simulink model "mux4_1_model"  (R2023b)
settings: Solver=VariableStepAuto  StartTime=0.0  StopTime=10.0  RelTol=1e-3
libraries: neural x204
(part 2 of 4)

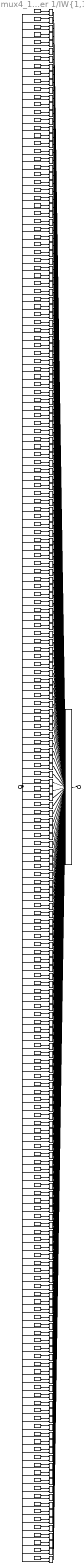
== system mux4_1_model/Pattern Recognition Neural Network/Layer 1/IW{1,1} ==
  "pd{1,1}" : Inport  PortDimensions=6
      mask Display: e = 0.06;c1 = [120 230 180]/255;c2 = ([120 230 180]+0)/(256+128);c3 = ([120 230 180]+128)/(256+128);patch([0 1 1 0],[0 0 1 1],c1);patch([0 1 1 1-e 1-e 0+e],[0 0 1 1-e 0+e 0+e],c2);patch([0 0 1 1-e 0+e 0+e],[0 1 1 1-e 1-e 0+e],c3);plot([0 1 1 0 0],[0 0 1 1 0]);
  "IW{1,1}(1,:)'" : Constant  Value=[1.88831465030217149347890881472267210483551025390625;-1.6328420936517591410819250086206011474132537841796875;-0.00712501113071774445917316853638112661428749561309814453125;0.95499304227647596743366875671199522912502288818359375;-0.8704765472023023864522883741301484405994415283203125;-1.8583799856878278067284782082424499094486236572265625]
      mask Display: e = 0.06;c1 = [120 150 230]/255;c2 = ([120 150 230]+0)/383;c3 = ([120 150 230]+128)/383;patch([0 1 1 0],[0 0 1 1],c1);patch([0 1 1 1-e 1-e 0+e],[0 0 1 1-e 0+e 0+e],c2);patch([0 0 1 1-e 0+e 0+e],[0 1 1 1-e 1-e 0+e],c3);plot([0 1 1 0 0],[0 0 1 1 0]);disp('Weights');
  "IW{1,1}(10,:)'" : Constant  Value=[-1.75938767476387436516915840911678969860076904296875;-1.1324850355018580838617481276742182672023773193359375;-2.119105979350400570382362275267951190471649169921875;0.50814743940664242050075927181751467287540435791015625;1.1338734712628728562577862248872406780719757080078125;-0.8131088091958151853333447434124536812305450439453125]
      mask Display: e = 0.06;c1 = [120 150 230]/255;c2 = ([120 150 230]+0)/383;c3 = ([120 150 230]+128)/383;patch([0 1 1 0],[0 0 1 1],c1);patch([0 1 1 1-e 1-e 0+e],[0 0 1 1-e 0+e 0+e],c2);patch([0 0 1 1-e 0+e 0+e],[0 1 1 1-e 1-e 0+e],c3);plot([0 1 1 0 0],[0 0 1 1 0]);disp('Weights');
  "IW{1,1}(100,:)'" : Constant  Value=[1.0766510821556865007408987366943620145320892333984375;2.50729854836723031752399037941358983516693115234375;-0.66792671741191711465290836713393218815326690673828125;1.2994231213573979033526484272442758083343505859375;-0.540478862160529871516700950451195240020751953125;-1.2539592132005139557549000528524629771709442138671875]
      mask Display: e = 0.06;c1 = [120 150 230]/255;c2 = ([120 150 230]+0)/383;c3 = ([120 150 230]+128)/383;patch([0 1 1 0],[0 0 1 1],c1);patch([0 1 1 1-e 1-e 0+e],[0 0 1 1-e 0+e 0+e],c2);patch([0 0 1 1-e 0+e 0+e],[0 1 1 1-e 1-e 0+e],c3);plot([0 1 1 0 0],[0 0 1 1 0]);disp('Weights');
  "IW{1,1}(101,:)'" : Constant  Value=[1.662379190191437761114912063931114971637725830078125;0.187490400635014820007739899665466509759426116943359375;-1.018279377777016492245820700190961360931396484375;-1.3995408467046546174827881259261630475521087646484375;-1.636461452276149142193162333569489419460296630859375;-1.73390509358015609819858582341112196445465087890625]
      mask Display: e = 0.06;c1 = [120 150 230]/255;c2 = ([120 150 230]+0)/383;c3 = ([120 150 230]+128)/383;patch([0 1 1 0],[0 0 1 1],c1);patch([0 1 1 1-e 1-e 0+e],[0 0 1 1-e 0+e 0+e],c2);patch([0 0 1 1-e 0+e 0+e],[0 1 1 1-e 1-e 0+e],c3);plot([0 1 1 0 0],[0 0 1 1 0]);disp('Weights');
  "IW{1,1}(102,:)'" : Constant  Value=[-1.3089337755879235647427094590966589748859405517578125;-1.9960191789693240149716757514397613704204559326171875;1.048776716022832733443692632135935127735137939453125;-1.4530345885058013610802163384505547583103179931640625;0.95098862747164381037379143890575505793094635009765625;1.3104674744980993050802453581127338111400604248046875]
      mask Display: e = 0.06;c1 = [120 150 230]/255;c2 = ([120 150 230]+0)/383;c3 = ([120 150 230]+128)/383;patch([0 1 1 0],[0 0 1 1],c1);patch([0 1 1 1-e 1-e 0+e],[0 0 1 1-e 0+e 0+e],c2);patch([0 0 1 1-e 0+e 0+e],[0 1 1 1-e 1-e 0+e],c3);plot([0 1 1 0 0],[0 0 1 1 0]);disp('Weights');
  "IW{1,1}(103,:)'" : Constant  Value=[2.034244858071051265113737827050499618053436279296875;-0.6838445544748481541574847142328508198261260986328125;0.31194926961552649213871291067334823310375213623046875;-0.9138731258806169766018001610063947737216949462890625;-2.21660641395503343886730363010428845882415771484375;-1.03046042192042275331687051220797002315521240234375]
      mask Display: e = 0.06;c1 = [120 150 230]/255;c2 = ([120 150 230]+0)/383;c3 = ([120 150 230]+128)/383;patch([0 1 1 0],[0 0 1 1],c1);patch([0 1 1 1-e 1-e 0+e],[0 0 1 1-e 0+e 0+e],c2);patch([0 0 1 1-e 0+e 0+e],[0 1 1 1-e 1-e 0+e],c3);plot([0 1 1 0 0],[0 0 1 1 0]);disp('Weights');
  "IW{1,1}(104,:)'" : Constant  Value=[1.2341260249343211086170413182117044925689697265625;1.9697753308339509548119394821696914732456207275390625;0.7954003142586156815951881071669049561023712158203125;-0.81498512744941986607472017567488364875316619873046875;-1.7842383912172545823437985745840705931186676025390625;1.27988877349261098714805484632961452007293701171875]
      mask Display: e = 0.06;c1 = [120 150 230]/255;c2 = ([120 150 230]+0)/383;c3 = ([120 150 230]+128)/383;patch([0 1 1 0],[0 0 1 1],c1);patch([0 1 1 1-e 1-e 0+e],[0 0 1 1-e 0+e 0+e],c2);patch([0 0 1 1-e 0+e 0+e],[0 1 1 1-e 1-e 0+e],c3);plot([0 1 1 0 0],[0 0 1 1 0]);disp('Weights');
  "IW{1,1}(105,:)'" : Constant  Value=[-0.6772763005036441796846702345646917819976806640625;-2.235366208999728154793729117955081164836883544921875;-1.664847534511748161634159259847365319728851318359375;1.1604986785562731999021934825577773153781890869140625;1.363475786119232591175887137069366872310638427734375;-0.038074786361743585827444036340239108540117740631103515625]
      mask Display: e = 0.06;c1 = [120 150 230]/255;c2 = ([120 150 230]+0)/383;c3 = ([120 150 230]+128)/383;patch([0 1 1 0],[0 0 1 1],c1);patch([0 1 1 1-e 1-e 0+e],[0 0 1 1-e 0+e 0+e],c2);patch([0 0 1 1-e 0+e 0+e],[0 1 1 1-e 1-e 0+e],c3);plot([0 1 1 0 0],[0 0 1 1 0]);disp('Weights');
  "IW{1,1}(106,:)'" : Constant  Value=[-1.0064124207377325159740166782285086810588836669921875;-1.85642466798463967592169865383766591548919677734375;0.51252403270238089394439384705037809908390045166015625;1.146135937560825102110584339243359863758087158203125;1.6304971971563133603666528870235197246074676513671875;-1.6941498966407813053791642232681624591350555419921875]
      mask Display: e = 0.06;c1 = [120 150 230]/255;c2 = ([120 150 230]+0)/383;c3 = ([120 150 230]+128)/383;patch([0 1 1 0],[0 0 1 1],c1);patch([0 1 1 1-e 1-e 0+e],[0 0 1 1-e 0+e 0+e],c2);patch([0 0 1 1-e 0+e 0+e],[0 1 1 1-e 1-e 0+e],c3);plot([0 1 1 0 0],[0 0 1 1 0]);disp('Weights');
  "IW{1,1}(107,:)'" : Constant  Value=[1.5111813479866660347994411495164968073368072509765625;-1.4606807787886146865474756850744597613811492919921875;0.30650959398300570146744803423644043505191802978515625;-0.31300585299283578688545048862579278647899627685546875;-1.6224966163979737121536572885815985500812530517578125;2.187239918452816400673555108369328081607818603515625]
      mask Display: e = 0.06;c1 = [120 150 230]/255;c2 = ([120 150 230]+0)/383;c3 = ([120 150 230]+128)/383;patch([0 1 1 0],[0 0 1 1],c1);patch([0 1 1 1-e 1-e 0+e],[0 0 1 1-e 0+e 0+e],c2);patch([0 0 1 1-e 0+e 0+e],[0 1 1 1-e 1-e 0+e],c3);plot([0 1 1 0 0],[0 0 1 1 0]);disp('Weights');
  "IW{1,1}(108,:)'" : Constant  Value=[-0.81530205261627630708431979655870236456394195556640625;0.670556113984504431613231645314954221248626708984375;2.113155561286254258135386407957412302494049072265625;1.2359534276509254180353991614538244903087615966796875;-1.87295706876884882063905024551786482334136962890625;-0.95610231061648665029650828728335909545421600341796875]
      mask Display: e = 0.06;c1 = [120 150 230]/255;c2 = ([120 150 230]+0)/383;c3 = ([120 150 230]+128)/383;patch([0 1 1 0],[0 0 1 1],c1);patch([0 1 1 1-e 1-e 0+e],[0 0 1 1-e 0+e 0+e],c2);patch([0 0 1 1-e 0+e 0+e],[0 1 1 1-e 1-e 0+e],c3);plot([0 1 1 0 0],[0 0 1 1 0]);disp('Weights');
  "IW{1,1}(109,:)'" : Constant  Value=[-0.436252319590053561082498845280497334897518157958984375;-0.09095977259585563690080789456260390579700469970703125;-2.019667451306033090219216319383122026920318603515625;1.135217226515316202295480252359993755817413330078125;-1.740452861528241523814131141989491879940032958984375;-1.719824326053439822459267816157080233097076416015625]
      mask Display: e = 0.06;c1 = [120 150 230]/255;c2 = ([120 150 230]+0)/383;c3 = ([120 150 230]+128)/383;patch([0 1 1 0],[0 0 1 1],c1);patch([0 1 1 1-e 1-e 0+e],[0 0 1 1-e 0+e 0+e],c2);patch([0 0 1 1-e 0+e 0+e],[0 1 1 1-e 1-e 0+e],c3);plot([0 1 1 0 0],[0 0 1 1 0]);disp('Weights');
  "IW{1,1}(11,:)'" : Constant  Value=[-1.86575481636632733994929367327131330966949462890625;0.259288778150366272523541510963696055114269256591796875;-1.8136703027089835504881421002210117876529693603515625;-0.91444566311584907225551432929933071136474609375;1.9041793386665977205751687506563030183315277099609375;-0.319398387228080171684752031069365330040454864501953125]
      mask Display: e = 0.06;c1 = [120 150 230]/255;c2 = ([120 150 230]+0)/383;c3 = ([120 150 230]+128)/383;patch([0 1 1 0],[0 0 1 1],c1);patch([0 1 1 1-e 1-e 0+e],[0 0 1 1-e 0+e 0+e],c2);patch([0 0 1 1-e 0+e 0+e],[0 1 1 1-e 1-e 0+e],c3);plot([0 1 1 0 0],[0 0 1 1 0]);disp('Weights');
  "IW{1,1}(110,:)'" : Constant  Value=[1.537058356646926693400700969505123794078826904296875;-0.9116668944426524756607932431506924331188201904296875;-1.3787755595316422141394241407397203147411346435546875;1.550419199126075842087857381557114422321319580078125;-1.0467684012883504696134195910417474806308746337890625;1.713054093403851840804463790846057236194610595703125]
      mask Display: e = 0.06;c1 = [120 150 230]/255;c2 = ([120 150 230]+0)/383;c3 = ([120 150 230]+128)/383;patch([0 1 1 0],[0 0 1 1],c1);patch([0 1 1 1-e 1-e 0+e],[0 0 1 1-e 0+e 0+e],c2);patch([0 0 1 1-e 0+e 0+e],[0 1 1 1-e 1-e 0+e],c3);plot([0 1 1 0 0],[0 0 1 1 0]);disp('Weights');
  "IW{1,1}(111,:)'" : Constant  Value=[-0.41550052784004432027131770155392587184906005859375;0.236723054659539633437503880486474372446537017822265625;1.7573231008430967303723946315585635602474212646484375;0.8226695216362298612722270263475365936756134033203125;-2.003254396611740428824077753233723342418670654296875;-1.9768638000240625895997936822823248803615570068359375]
      mask Display: e = 0.06;c1 = [120 150 230]/255;c2 = ([120 150 230]+0)/383;c3 = ([120 150 230]+128)/383;patch([0 1 1 0],[0 0 1 1],c1);patch([0 1 1 1-e 1-e 0+e],[0 0 1 1-e 0+e 0+e],c2);patch([0 0 1 1-e 0+e 0+e],[0 1 1 1-e 1-e 0+e],c3);plot([0 1 1 0 0],[0 0 1 1 0]);disp('Weights');
  "IW{1,1}(112,:)'" : Constant  Value=[-0.1553479606238077348479009742732159793376922607421875;0.70635925505895313936122192899347282946109771728515625;0.034497490565917721117017435972229577600955963134765625;-1.6002764274101297647945330027141608297824859619140625;-1.86061865188189567987819827976636588573455810546875;2.3375659489914095701124097104184329509735107421875]
      mask Display: e = 0.06;c1 = [120 150 230]/255;c2 = ([120 150 230]+0)/383;c3 = ([120 150 230]+128)/383;patch([0 1 1 0],[0 0 1 1],c1);patch([0 1 1 1-e 1-e 0+e],[0 0 1 1-e 0+e 0+e],c2);patch([0 0 1 1-e 0+e 0+e],[0 1 1 1-e 1-e 0+e],c3);plot([0 1 1 0 0],[0 0 1 1 0]);disp('Weights');
  "IW{1,1}(113,:)'" : Constant  Value=[-1.845377127149288920548997339210473001003265380859375;1.361228310922412365613354268134571611881256103515625;-0.758660517597993244720555594540201127529144287109375;-1.6822874639743139457692677751765586435794830322265625;1.095563177245159725003986750380136072635650634765625;-1.1994489528488203600176120744436047971248626708984375]
      mask Display: e = 0.06;c1 = [120 150 230]/255;c2 = ([120 150 230]+0)/383;c3 = ([120 150 230]+128)/383;patch([0 1 1 0],[0 0 1 1],c1);patch([0 1 1 1-e 1-e 0+e],[0 0 1 1-e 0+e 0+e],c2);patch([0 0 1 1-e 0+e 0+e],[0 1 1 1-e 1-e 0+e],c3);plot([0 1 1 0 0],[0 0 1 1 0]);disp('Weights');
  "IW{1,1}(114,:)'" : Constant  Value=[-1.1532348209103002734110532401246018707752227783203125;2.02574040678284550409671282977797091007232666015625;0.03595926287364765994158943840375286526978015899658203125;1.637336374892405910230763765866868197917938232421875;-1.4152723289234547809911646254477091133594512939453125;-1.342590343662893648257750101038254797458648681640625]
      mask Display: e = 0.06;c1 = [120 150 230]/255;c2 = ([120 150 230]+0)/383;c3 = ([120 150 230]+128)/383;patch([0 1 1 0],[0 0 1 1],c1);patch([0 1 1 1-e 1-e 0+e],[0 0 1 1-e 0+e 0+e],c2);patch([0 0 1 1-e 0+e 0+e],[0 1 1 1-e 1-e 0+e],c3);plot([0 1 1 0 0],[0 0 1 1 0]);disp('Weights');
  "IW{1,1}(115,:)'" : Constant  Value=[-1.5524401238853666740169501281343400478363037109375;1.666216443357559029436743003316223621368408203125;-1.082598303285360774594892063760198652744293212890625;-0.81942242561225320240936298432643525302410125732421875;-0.7656941750687067393954521321575157344341278076171875;1.9201958846802698044342605498968623578548431396484375]
      mask Display: e = 0.06;c1 = [120 150 230]/255;c2 = ([120 150 230]+0)/383;c3 = ([120 150 230]+128)/383;patch([0 1 1 0],[0 0 1 1],c1);patch([0 1 1 1-e 1-e 0+e],[0 0 1 1-e 0+e 0+e],c2);patch([0 0 1 1-e 0+e 0+e],[0 1 1 1-e 1-e 0+e],c3);plot([0 1 1 0 0],[0 0 1 1 0]);disp('Weights');
  "IW{1,1}(116,:)'" : Constant  Value=[-1.7401694103994957973924329053261317312717437744140625;1.47612141184980760755252049420960247516632080078125;-0.8518124355427427740750090379151515662670135498046875;1.5173408084150123986688640798092819750308990478515625;-0.72172092986768487943294303477159701287746429443359375;1.5888961206524860880762162196333520114421844482421875]
      mask Display: e = 0.06;c1 = [120 150 230]/255;c2 = ([120 150 230]+0)/383;c3 = ([120 150 230]+128)/383;patch([0 1 1 0],[0 0 1 1],c1);patch([0 1 1 1-e 1-e 0+e],[0 0 1 1-e 0+e 0+e],c2);patch([0 0 1 1-e 0+e 0+e],[0 1 1 1-e 1-e 0+e],c3);plot([0 1 1 0 0],[0 0 1 1 0]);disp('Weights');
  "IW{1,1}(117,:)'" : Constant  Value=[-1.899523414272333621255484104040078818798065185546875;0.155841010708632043968435709757613949477672576904296875;-2.08942613232541329892910653143189847469329833984375;1.6325415730440149264524052341585047543048858642578125;0.269439984105174501483048743466497398912906646728515625;0.8416068349956320471250137416063807904720306396484375]
      mask Display: e = 0.06;c1 = [120 150 230]/255;c2 = ([120 150 230]+0)/383;c3 = ([120 150 230]+128)/383;patch([0 1 1 0],[0 0 1 1],c1);patch([0 1 1 1-e 1-e 0+e],[0 0 1 1-e 0+e 0+e],c2);patch([0 0 1 1-e 0+e 0+e],[0 1 1 1-e 1-e 0+e],c3);plot([0 1 1 0 0],[0 0 1 1 0]);disp('Weights');
  "IW{1,1}(118,:)'" : Constant  Value=[-0.87634837696015266406135424404055811464786529541015625;-1.7801798972276754451371516552171669900417327880859375;2.0552891938640858171538638998754322528839111328125;-1.6794680704590005948517728029401041567325592041015625;-0.015750101229376957390204694320345879532396793365478515625;0.8263635683078442983884315253817476332187652587890625]
      mask Display: e = 0.06;c1 = [120 150 230]/255;c2 = ([120 150 230]+0)/383;c3 = ([120 150 230]+128)/383;patch([0 1 1 0],[0 0 1 1],c1);patch([0 1 1 1-e 1-e 0+e],[0 0 1 1-e 0+e 0+e],c2);patch([0 0 1 1-e 0+e 0+e],[0 1 1 1-e 1-e 0+e],c3);plot([0 1 1 0 0],[0 0 1 1 0]);disp('Weights');
  "IW{1,1}(119,:)'" : Constant  Value=[-1.516871482482184063655950012616813182830810546875;0.2370260290232108213448469768991344608366489410400390625;0.3801253712942063156532412904198281466960906982421875;2.412357471952862653097326983697712421417236328125;1.507165727561675883094949313090182840824127197265625;-0.929618773510952678407193161547183990478515625]
      mask Display: e = 0.06;c1 = [120 150 230]/255;c2 = ([120 150 230]+0)/383;c3 = ([120 150 230]+128)/383;patch([0 1 1 0],[0 0 1 1],c1);patch([0 1 1 1-e 1-e 0+e],[0 0 1 1-e 0+e 0+e],c2);patch([0 0 1 1-e 0+e 0+e],[0 1 1 1-e 1-e 0+e],c3);plot([0 1 1 0 0],[0 0 1 1 0]);disp('Weights');
  "IW{1,1}(12,:)'" : Constant  Value=[-0.09285344453561028554844369864440523087978363037109375;-0.1842082224482888275218783746822737157344818115234375;-2.073360096033266319892618412268348038196563720703125;-2.4221605191648567512174849980510771274566650390625;1.0905367265629186679376516622141934931278228759765625;-0.1863687345116258331501057909918017685413360595703125]
      mask Display: e = 0.06;c1 = [120 150 230]/255;c2 = ([120 150 230]+0)/383;c3 = ([120 150 230]+128)/383;patch([0 1 1 0],[0 0 1 1],c1);patch([0 1 1 1-e 1-e 0+e],[0 0 1 1-e 0+e 0+e],c2);patch([0 0 1 1-e 0+e 0+e],[0 1 1 1-e 1-e 0+e],c3);plot([0 1 1 0 0],[0 0 1 1 0]);disp('Weights');
  "IW{1,1}(120,:)'" : Constant  Value=[0.7298760298497335430312205062364228069782257080078125;1.7054105885259678299092911402112804353237152099609375;-1.3051263069442622377636098462971858680248260498046875;-1.35858548608056661777254703338257968425750732421875;1.917274474423834806913191641797311604022979736328125;0.86507265992183801639470175359747372567653656005859375]
      mask Display: e = 0.06;c1 = [120 150 230]/255;c2 = ([120 150 230]+0)/383;c3 = ([120 150 230]+128)/383;patch([0 1 1 0],[0 0 1 1],c1);patch([0 1 1 1-e 1-e 0+e],[0 0 1 1-e 0+e 0+e],c2);patch([0 0 1 1-e 0+e 0+e],[0 1 1 1-e 1-e 0+e],c3);plot([0 1 1 0 0],[0 0 1 1 0]);disp('Weights');
  "IW{1,1}(121,:)'" : Constant  Value=[-0.73181033977736176243666932350606657564640045166015625;0.312391685715092071173870635902858339250087738037109375;-0.0668938432206781230515701963668107055127620697021484375;2.07913361094917892302191830822266638278961181640625;-2.520514999819232659916679040179587900638580322265625;-0.146896648267278440158634111867286264896392822265625]
      mask Display: e = 0.06;c1 = [120 150 230]/255;c2 = ([120 150 230]+0)/383;c3 = ([120 150 230]+128)/383;patch([0 1 1 0],[0 0 1 1],c1);patch([0 1 1 1-e 1-e 0+e],[0 0 1 1-e 0+e 0+e],c2);patch([0 0 1 1-e 0+e 0+e],[0 1 1 1-e 1-e 0+e],c3);plot([0 1 1 0 0],[0 0 1 1 0]);disp('Weights');
  "IW{1,1}(122,:)'" : Constant  Value=[1.3070750508070141382432893806253559887409210205078125;-0.9616164029817337866035131810349412262439727783203125;-0.08443827552280382120475366036771447397768497467041015625;2.193825628303860408863101838505826890468597412109375;1.52403626309709494535127305425703525543212890625;-1.309713213829291955647704526199959218502044677734375]
      mask Display: e = 0.06;c1 = [120 150 230]/255;c2 = ([120 150 230]+0)/383;c3 = ([120 150 230]+128)/383;patch([0 1 1 0],[0 0 1 1],c1);patch([0 1 1 1-e 1-e 0+e],[0 0 1 1-e 0+e 0+e],c2);patch([0 0 1 1-e 0+e 0+e],[0 1 1 1-e 1-e 0+e],c3);plot([0 1 1 0 0],[0 0 1 1 0]);disp('Weights');
  "IW{1,1}(123,:)'" : Constant  Value=[-1.49923712543691944887314093648456037044525146484375;0.4244620066469833030708969090483151376247406005859375;-0.40272808530360026946226525979000143706798553466796875;-1.5141286090609884507074411885696463286876678466796875;-2.359891218442819127432130699162371456623077392578125;-1.0018908630430416462075982053647749125957489013671875]
      mask Display: e = 0.06;c1 = [120 150 230]/255;c2 = ([120 150 230]+0)/383;c3 = ([120 150 230]+128)/383;patch([0 1 1 0],[0 0 1 1],c1);patch([0 1 1 1-e 1-e 0+e],[0 0 1 1-e 0+e 0+e],c2);patch([0 0 1 1-e 0+e 0+e],[0 1 1 1-e 1-e 0+e],c3);plot([0 1 1 0 0],[0 0 1 1 0]);disp('Weights');
  "IW{1,1}(124,:)'" : Constant  Value=[1.5322902368928794647473523582448251545429229736328125;-0.11793400773590911878585529848351143300533294677734375;-0.6851081461647317016883107498870231211185455322265625;-0.2943333478712519823972115773358382284641265869140625;2.505058700623063128176681857439689338207244873046875;-1.5812466947481340628911539170076139271259307861328125]
      mask Display: e = 0.06;c1 = [120 150 230]/255;c2 = ([120 150 230]+0)/383;c3 = ([120 150 230]+128)/383;patch([0 1 1 0],[0 0 1 1],c1);patch([0 1 1 1-e 1-e 0+e],[0 0 1 1-e 0+e 0+e],c2);patch([0 0 1 1-e 0+e 0+e],[0 1 1 1-e 1-e 0+e],c3);plot([0 1 1 0 0],[0 0 1 1 0]);disp('Weights');
  "IW{1,1}(125,:)'" : Constant  Value=[-2.68677738690151812761541805230081081390380859375;-1.5401660115698267983219693633145652711391448974609375;-0.32853506182747749253536539981723763048648834228515625;0.9283880104413213540937022116850130259990692138671875;0.04234698018822520559911737336733494885265827178955078125;0.9995731367004336842541079022339545190334320068359375]
      mask Display: e = 0.06;c1 = [120 150 230]/255;c2 = ([120 150 230]+0)/383;c3 = ([120 150 230]+128)/383;patch([0 1 1 0],[0 0 1 1],c1);patch([0 1 1 1-e 1-e 0+e],[0 0 1 1-e 0+e 0+e],c2);patch([0 0 1 1-e 0+e 0+e],[0 1 1 1-e 1-e 0+e],c3);plot([0 1 1 0 0],[0 0 1 1 0]);disp('Weights');
  "IW{1,1}(126,:)'" : Constant  Value=[0.457656071818612841806128699317923747003078460693359375;2.265153444827204598510661526233889162540435791015625;0.95669467375376660012165075386292301118373870849609375;-0.096484289563831648894876025224220938980579376220703125;-1.3548035008472638640597551784594543278217315673828125;-1.9258228536002415243189034299575723707675933837890625]
      mask Display: e = 0.06;c1 = [120 150 230]/255;c2 = ([120 150 230]+0)/383;c3 = ([120 150 230]+128)/383;patch([0 1 1 0],[0 0 1 1],c1);patch([0 1 1 1-e 1-e 0+e],[0 0 1 1-e 0+e 0+e],c2);patch([0 0 1 1-e 0+e 0+e],[0 1 1 1-e 1-e 0+e],c3);plot([0 1 1 0 0],[0 0 1 1 0]);disp('Weights');
  "IW{1,1}(127,:)'" : Constant  Value=[-0.75665291597339001672395397690706886351108551025390625;1.9028383927140042342074366388260386884212493896484375;-0.2233557391700828620439978067224728874862194061279296875;-1.5112287486513700240919888528878800570964813232421875;-1.690661519385519451219579423195682466030120849609375;1.420623507139258112630386676755733788013458251953125]
      mask Display: e = 0.06;c1 = [120 150 230]/255;c2 = ([120 150 230]+0)/383;c3 = ([120 150 230]+128)/383;patch([0 1 1 0],[0 0 1 1],c1);patch([0 1 1 1-e 1-e 0+e],[0 0 1 1-e 0+e 0+e],c2);patch([0 0 1 1-e 0+e 0+e],[0 1 1 1-e 1-e 0+e],c3);plot([0 1 1 0 0],[0 0 1 1 0]);disp('Weights');
  "IW{1,1}(128,:)'" : Constant  Value=[-1.44129992615077551221247631474398076534271240234375;1.4293269426266572708072999375872313976287841796875;-2.19625833799338199270323457312770187854766845703125;0.83262127728390888936615965576493181288242340087890625;-1.0087616431711523556913334687124006450176239013671875;-0.77970252370232373539948866891791112720966339111328125]
      mask Display: e = 0.06;c1 = [120 150 230]/255;c2 = ([120 150 230]+0)/383;c3 = ([120 150 230]+128)/383;patch([0 1 1 0],[0 0 1 1],c1);patch([0 1 1 1-e 1-e 0+e],[0 0 1 1-e 0+e 0+e],c2);patch([0 0 1 1-e 0+e 0+e],[0 1 1 1-e 1-e 0+e],c3);plot([0 1 1 0 0],[0 0 1 1 0]);disp('Weights');
  "IW{1,1}(129,:)'" : Constant  Value=[-2.0977566009598209717523786821402609348297119140625;1.0927019132808697410297327223815955221652984619140625;-1.0054952010366411396802277522510848939418792724609375;-0.79642250791848656632510028430260717868804931640625;-1.93440528265185918144197785295546054840087890625;0.904870480070645299974785302765667438507080078125]
      mask Display: e = 0.06;c1 = [120 150 230]/255;c2 = ([120 150 230]+0)/383;c3 = ([120 150 230]+128)/383;patch([0 1 1 0],[0 0 1 1],c1);patch([0 1 1 1-e 1-e 0+e],[0 0 1 1-e 0+e 0+e],c2);patch([0 0 1 1-e 0+e 0+e],[0 1 1 1-e 1-e 0+e],c3);plot([0 1 1 0 0],[0 0 1 1 0]);disp('Weights');
  "IW{1,1}(13,:)'" : Constant  Value=[2.091769591013599605133777004084549844264984130859375;0.41385057928697255302807889165706001222133636474609375;1.989760868931273574133911097305826842784881591796875;1.4398635501659773350269233560538850724697113037109375;0.8120504378848452109451727665145881474018096923828125;0.292866351433269500592615486311842687427997589111328125]
      mask Display: e = 0.06;c1 = [120 150 230]/255;c2 = ([120 150 230]+0)/383;c3 = ([120 150 230]+128)/383;patch([0 1 1 0],[0 0 1 1],c1);patch([0 1 1 1-e 1-e 0+e],[0 0 1 1-e 0+e 0+e],c2);patch([0 0 1 1-e 0+e 0+e],[0 1 1 1-e 1-e 0+e],c3);plot([0 1 1 0 0],[0 0 1 1 0]);disp('Weights');
  "IW{1,1}(130,:)'" : Constant  Value=[1.642323168220304996367531202849932014942169189453125;1.6715915844030515557960825390182435512542724609375;0.07189659407978006566697359858153504319489002227783203125;0.71205568209645597743673306467826478183269500732421875;1.480426424780183491947127549792639911174774169921875;1.7738718406404625493877347253146581351757049560546875]
      mask Display: e = 0.06;c1 = [120 150 230]/255;c2 = ([120 150 230]+0)/383;c3 = ([120 150 230]+128)/383;patch([0 1 1 0],[0 0 1 1],c1);patch([0 1 1 1-e 1-e 0+e],[0 0 1 1-e 0+e 0+e],c2);patch([0 0 1 1-e 0+e 0+e],[0 1 1 1-e 1-e 0+e],c3);plot([0 1 1 0 0],[0 0 1 1 0]);disp('Weights');
  "IW{1,1}(131,:)'" : Constant  Value=[1.1561621493425373596863892089459113776683807373046875;0.70996729571562033900278265718952752649784088134765625;0.65702249406333346204434064929955638945102691650390625;1.7389816541611187172833297154284082353115081787109375;-1.6145127293904806276003682796726934611797332763671875;1.8873230443673689737948961919755674898624420166015625]
      mask Display: e = 0.06;c1 = [120 150 230]/255;c2 = ([120 150 230]+0)/383;c3 = ([120 150 230]+128)/383;patch([0 1 1 0],[0 0 1 1],c1);patch([0 1 1 1-e 1-e 0+e],[0 0 1 1-e 0+e 0+e],c2);patch([0 0 1 1-e 0+e 0+e],[0 1 1 1-e 1-e 0+e],c3);plot([0 1 1 0 0],[0 0 1 1 0]);disp('Weights');
  "IW{1,1}(132,:)'" : Constant  Value=[1.3500591886800383800704139503068290650844573974609375;-1.66564321719388797049532513483427464962005615234375;-0.86416547251374209448471219729981385171413421630859375;0.418297532000039662403167994852992706000804901123046875;-0.636674882782167106398674150113947689533233642578125;2.29176104609416864121840262669138610363006591796875]
      mask Display: e = 0.06;c1 = [120 150 230]/255;c2 = ([120 150 230]+0)/383;c3 = ([120 150 230]+128)/383;patch([0 1 1 0],[0 0 1 1],c1);patch([0 1 1 1-e 1-e 0+e],[0 0 1 1-e 0+e 0+e],c2);patch([0 0 1 1-e 0+e 0+e],[0 1 1 1-e 1-e 0+e],c3);plot([0 1 1 0 0],[0 0 1 1 0]);disp('Weights');
  "IW{1,1}(133,:)'" : Constant  Value=[1.7562502929443386534558158018626272678375244140625;1.4179403797342262638636611882247962057590484619140625;-0.58888339131365607936885453455033712089061737060546875;-1.5084478552824738262216897055623121559619903564453125;-1.368012614763485235158668729127384722232818603515625;1.329596182580093710612345603294670581817626953125]
      mask Display: e = 0.06;c1 = [120 150 230]/255;c2 = ([120 150 230]+0)/383;c3 = ([120 150 230]+128)/383;patch([0 1 1 0],[0 0 1 1],c1);patch([0 1 1 1-e 1-e 0+e],[0 0 1 1-e 0+e 0+e],c2);patch([0 0 1 1-e 0+e 0+e],[0 1 1 1-e 1-e 0+e],c3);plot([0 1 1 0 0],[0 0 1 1 0]);disp('Weights');
  "IW{1,1}(134,:)'" : Constant  Value=[-1.058495654154327336726737485150806605815887451171875;-1.4114962887591586682134447983116842806339263916015625;-2.220444979734403911919571328326128423213958740234375;0.372784392207425152587774164203437976539134979248046875;1.7349297171019502084021723931073211133480072021484375;-0.6071887885852900179628477417281828820705413818359375]
      mask Display: e = 0.06;c1 = [120 150 230]/255;c2 = ([120 150 230]+0)/383;c3 = ([120 150 230]+128)/383;patch([0 1 1 0],[0 0 1 1],c1);patch([0 1 1 1-e 1-e 0+e],[0 0 1 1-e 0+e 0+e],c2);patch([0 0 1 1-e 0+e 0+e],[0 1 1 1-e 1-e 0+e],c3);plot([0 1 1 0 0],[0 0 1 1 0]);disp('Weights');
  "IW{1,1}(135,:)'" : Constant  Value=[-0.92881518491902903544854552819742821156978607177734375;2.063776476347365385066723320051096379756927490234375;1.115820184186749219890089079854078590869903564453125;1.88853050385999399196634840336628258228302001953125;-0.64429482327307907585378643489093519747257232666015625;-1.10686921874346300143088228651322424411773681640625]
      mask Display: e = 0.06;c1 = [120 150 230]/255;c2 = ([120 150 230]+0)/383;c3 = ([120 150 230]+128)/383;patch([0 1 1 0],[0 0 1 1],c1);patch([0 1 1 1-e 1-e 0+e],[0 0 1 1-e 0+e 0+e],c2);patch([0 0 1 1-e 0+e 0+e],[0 1 1 1-e 1-e 0+e],c3);plot([0 1 1 0 0],[0 0 1 1 0]);disp('Weights');
  "IW{1,1}(136,:)'" : Constant  Value=[2.036609164391787629710961482487618923187255859375;-0.1280157127676240513824978961565648205578327178955078125;-0.263202182254216487944376012819702737033367156982421875;-0.79729874233306385900021950874361209571361541748046875;2.543881563311895632750747608952224254608154296875;-0.30282514188475440075620781499310396611690521240234375]
      mask Display: e = 0.06;c1 = [120 150 230]/255;c2 = ([120 150 230]+0)/383;c3 = ([120 150 230]+128)/383;patch([0 1 1 0],[0 0 1 1],c1);patch([0 1 1 1-e 1-e 0+e],[0 0 1 1-e 0+e 0+e],c2);patch([0 0 1 1-e 0+e 0+e],[0 1 1 1-e 1-e 0+e],c3);plot([0 1 1 0 0],[0 0 1 1 0]);disp('Weights');
  "IW{1,1}(137,:)'" : Constant  Value=[-0.5037815361707365102716948968009091913700103759765625;0.815746113997100952275332019780762493610382080078125;0.38447320404987639363980633788742125034332275390625;2.3893817298616593092219773097895085811614990234375;-2.083522374996051862439117030589841306209564208984375;-0.4991731637154857015303832667996175587177276611328125]
      mask Display: e = 0.06;c1 = [120 150 230]/255;c2 = ([120 150 230]+0)/383;c3 = ([120 150 230]+128)/383;patch([0 1 1 0],[0 0 1 1],c1);patch([0 1 1 1-e 1-e 0+e],[0 0 1 1-e 0+e 0+e],c2);patch([0 0 1 1-e 0+e 0+e],[0 1 1 1-e 1-e 0+e],c3);plot([0 1 1 0 0],[0 0 1 1 0]);disp('Weights');
  "IW{1,1}(138,:)'" : Constant  Value=[-0.1461107710609940435464437769041978754103183746337890625;1.1830069221112140542828683464904315769672393798828125;0.34958795177155665978574461405514739453792572021484375;-3.12225419745804888549400857300497591495513916015625;0.3209669389391738292260924936272203922271728515625;-0.28800515491499112386009073816239833831787109375]
      mask Display: e = 0.06;c1 = [120 150 230]/255;c2 = ([120 150 230]+0)/383;c3 = ([120 150 230]+128)/383;patch([0 1 1 0],[0 0 1 1],c1);patch([0 1 1 1-e 1-e 0+e],[0 0 1 1-e 0+e 0+e],c2);patch([0 0 1 1-e 0+e 0+e],[0 1 1 1-e 1-e 0+e],c3);plot([0 1 1 0 0],[0 0 1 1 0]);disp('Weights');
  "IW{1,1}(139,:)'" : Constant  Value=[1.1617009772980677606568633564165793359279632568359375;-2.081156082091216941165612297481857240200042724609375;0.6929679164687405634737160653457976877689361572265625;0.09026726970409222616797961791235138662159442901611328125;-1.619637926752290457699245962430723011493682861328125;-1.8956215286323845337079774253652431070804595947265625]
      mask Display: e = 0.06;c1 = [120 150 230]/255;c2 = ([120 150 230]+0)/383;c3 = ([120 150 230]+128)/383;patch([0 1 1 0],[0 0 1 1],c1);patch([0 1 1 1-e 1-e 0+e],[0 0 1 1-e 0+e 0+e],c2);patch([0 0 1 1-e 0+e 0+e],[0 1 1 1-e 1-e 0+e],c3);plot([0 1 1 0 0],[0 0 1 1 0]);disp('Weights');
  "IW{1,1}(14,:)'" : Constant  Value=[0.130370910445221699358597788886982016265392303466796875;0.06595470879224892002401503532382776029407978057861328125;0.93778329616634292786869764313451014459133148193359375;-2.06969875084817456212249453528784215450286865234375;1.4934974278543702297383788391016423702239990234375;1.88755523690793847180202646995894610881805419921875]
      mask Display: e = 0.06;c1 = [120 150 230]/255;c2 = ([120 150 230]+0)/383;c3 = ([120 150 230]+128)/383;patch([0 1 1 0],[0 0 1 1],c1);patch([0 1 1 1-e 1-e 0+e],[0 0 1 1-e 0+e 0+e],c2);patch([0 0 1 1-e 0+e 0+e],[0 1 1 1-e 1-e 0+e],c3);plot([0 1 1 0 0],[0 0 1 1 0]);disp('Weights');
  "IW{1,1}(140,:)'" : Constant  Value=[-1.5668111318511872553926878026686608791351318359375;-1.8963900555458652608109559878357686102390289306640625;-0.09058730954043255068075524150117416866123676300048828125;2.00894296069608646604365276289172470569610595703125;-1.1076115689669041586284947698004543781280517578125;-0.68337109145663121889668900621472857892513275146484375]
      mask Display: e = 0.06;c1 = [120 150 230]/255;c2 = ([120 150 230]+0)/383;c3 = ([120 150 230]+128)/383;patch([0 1 1 0],[0 0 1 1],c1);patch([0 1 1 1-e 1-e 0+e],[0 0 1 1-e 0+e 0+e],c2);patch([0 0 1 1-e 0+e 0+e],[0 1 1 1-e 1-e 0+e],c3);plot([0 1 1 0 0],[0 0 1 1 0]);disp('Weights');
  "IW{1,1}(141,:)'" : Constant  Value=[-0.493181477548115976272669058744213543832302093505859375;-1.5325804228412633900546779841533862054347991943359375;-2.771100199064796765213714024866931140422821044921875;-0.057448910909267451863069453565913136117160320281982421875;0.86324146711337246262729649970424361526966094970703125;-0.85581749069124446460676836068159900605678558349609375]
      mask Display: e = 0.06;c1 = [120 150 230]/255;c2 = ([120 150 230]+0)/383;c3 = ([120 150 230]+128)/383;patch([0 1 1 0],[0 0 1 1],c1);patch([0 1 1 1-e 1-e 0+e],[0 0 1 1-e 0+e 0+e],c2);patch([0 0 1 1-e 0+e 0+e],[0 1 1 1-e 1-e 0+e],c3);plot([0 1 1 0 0],[0 0 1 1 0]);disp('Weights');
  "IW{1,1}(142,:)'" : Constant  Value=[-1.197002594050322610286229974008165299892425537109375;-2.06012164904401284815094186342321336269378662109375;-0.55514828096147506020230366630130447447299957275390625;-0.72939387634823338313339036176330409944057464599609375;2.17964632194250729213536033057607710361480712890625;-0.331769298810621615647420412642532028257846832275390625]
      mask Display: e = 0.06;c1 = [120 150 230]/255;c2 = ([120 150 230]+0)/383;c3 = ([120 150 230]+128)/383;patch([0 1 1 0],[0 0 1 1],c1);patch([0 1 1 1-e 1-e 0+e],[0 0 1 1-e 0+e 0+e],c2);patch([0 0 1 1-e 0+e 0+e],[0 1 1 1-e 1-e 0+e],c3);plot([0 1 1 0 0],[0 0 1 1 0]);disp('Weights');
  "IW{1,1}(143,:)'" : Constant  Value=[-1.89530879134973506694450406939722597599029541015625;0.78522114584999991304670174940838478505611419677734375;-1.62981252929749498292721909820102155208587646484375;-0.0217639011993176027803809091665243613533675670623779296875;1.4427206524186149128041734002181328833103179931640625;-1.6263689841685760040235209089587442576885223388671875]
      mask Display: e = 0.06;c1 = [120 150 230]/255;c2 = ([120 150 230]+0)/383;c3 = ([120 150 230]+128)/383;patch([0 1 1 0],[0 0 1 1],c1);patch([0 1 1 1-e 1-e 0+e],[0 0 1 1-e 0+e 0+e],c2);patch([0 0 1 1-e 0+e 0+e],[0 1 1 1-e 1-e 0+e],c3);plot([0 1 1 0 0],[0 0 1 1 0]);disp('Weights');
  "IW{1,1}(144,:)'" : Constant  Value=[1.8842090238854665162904211683780886232852935791015625;-0.6075292780804424364049509676988236606121063232421875;-1.9113951015001158229011934963637031614780426025390625;0.0974919111882766864507487980517907999455928802490234375;1.9049949416639415655794209669693373143672943115234375;0.724713253659541312146075142663903534412384033203125]
      mask Display: e = 0.06;c1 = [120 150 230]/255;c2 = ([120 150 230]+0)/383;c3 = ([120 150 230]+128)/383;patch([0 1 1 0],[0 0 1 1],c1);patch([0 1 1 1-e 1-e 0+e],[0 0 1 1-e 0+e 0+e],c2);patch([0 0 1 1-e 0+e 0+e],[0 1 1 1-e 1-e 0+e],c3);plot([0 1 1 0 0],[0 0 1 1 0]);disp('Weights');
  "IW{1,1}(145,:)'" : Constant  Value=[0.41305865362062810230980858250404708087444305419921875;0.356846198652678359142242925372556783258914947509765625;-1.2114844952700967173342405658331699669361114501953125;2.045676916575862147595898932195268571376800537109375;0.741817205974896420883624159614555537700653076171875;-2.263235575806954447131147389882244169712066650390625]
      mask Display: e = 0.06;c1 = [120 150 230]/255;c2 = ([120 150 230]+0)/383;c3 = ([120 150 230]+128)/383;patch([0 1 1 0],[0 0 1 1],c1);patch([0 1 1 1-e 1-e 0+e],[0 0 1 1-e 0+e 0+e],c2);patch([0 0 1 1-e 0+e 0+e],[0 1 1 1-e 1-e 0+e],c3);plot([0 1 1 0 0],[0 0 1 1 0]);disp('Weights');
  "IW{1,1}(146,:)'" : Constant  Value=[-0.9008574792966952404782432495267130434513092041015625;-2.319392326746150700955695356242358684539794921875;-1.055815889789439854240526983630843460559844970703125;-1.0826923083773867251267120082047767937183380126953125;0.420690200351257315158903793417266570031642913818359375;1.71475202633863954559956255252473056316375732421875]
      mask Display: e = 0.06;c1 = [120 150 230]/255;c2 = ([120 150 230]+0)/383;c3 = ([120 150 230]+128)/383;patch([0 1 1 0],[0 0 1 1],c1);patch([0 1 1 1-e 1-e 0+e],[0 0 1 1-e 0+e 0+e],c2);patch([0 0 1 1-e 0+e 0+e],[0 1 1 1-e 1-e 0+e],c3);plot([0 1 1 0 0],[0 0 1 1 0]);disp('Weights');
  "IW{1,1}(147,:)'" : Constant  Value=[-1.8657348896215013578370189861743710935115814208984375;-1.808173279651605458440144502674229443073272705078125;-1.356709286650181756073152428143657743930816650390625;0.6217501894101615800281024348805658519268035888671875;1.238465600404463629047313588671386241912841796875;-0.9240999480794018783313958920189179480075836181640625]
      mask Display: e = 0.06;c1 = [120 150 230]/255;c2 = ([120 150 230]+0)/383;c3 = ([120 150 230]+128)/383;patch([0 1 1 0],[0 0 1 1],c1);patch([0 1 1 1-e 1-e 0+e],[0 0 1 1-e 0+e 0+e],c2);patch([0 0 1 1-e 0+e 0+e],[0 1 1 1-e 1-e 0+e],c3);plot([0 1 1 0 0],[0 0 1 1 0]);disp('Weights');
  "IW{1,1}(148,:)'" : Constant  Value=[1.3273967969385098708556824931292794644832611083984375;1.602140748976784490054114939994178712368011474609375;2.355541506071918700371270460891537368297576904296875;0.5700044310759844190528156104846857488155364990234375;-0.95792229277017149069450852039153687655925750732421875;-0.03538063002234291543057764783952734433114528656005859375]
      mask Display: e = 0.06;c1 = [120 150 230]/255;c2 = ([120 150 230]+0)/383;c3 = ([120 150 230]+128)/383;patch([0 1 1 0],[0 0 1 1],c1);patch([0 1 1 1-e 1-e 0+e],[0 0 1 1-e 0+e 0+e],c2);patch([0 0 1 1-e 0+e 0+e],[0 1 1 1-e 1-e 0+e],c3);plot([0 1 1 0 0],[0 0 1 1 0]);disp('Weights');
  "IW{1,1}(149,:)'" : Constant  Value=[1.823832672938071386425917808082886040210723876953125;-1.7778507285522879843853161219158209860324859619140625;0.40863846088071842377331677198526449501514434814453125;-1.025007037315884161898793536238372325897216796875;1.140130686179925856293948527309112250804901123046875;-1.55655716652775932828944860375486314296722412109375]
      mask Display: e = 0.06;c1 = [120 150 230]/255;c2 = ([120 150 230]+0)/383;c3 = ([120 150 230]+128)/383;patch([0 1 1 0],[0 0 1 1],c1);patch([0 1 1 1-e 1-e 0+e],[0 0 1 1-e 0+e 0+e],c2);patch([0 0 1 1-e 0+e 0+e],[0 1 1 1-e 1-e 0+e],c3);plot([0 1 1 0 0],[0 0 1 1 0]);disp('Weights');
  "IW{1,1}(15,:)'" : Constant  Value=[-1.324881363200605566277090474613942205905914306640625;1.1536904791992099728048515316913835704326629638671875;-1.6016606635338386244171715588890947401523590087890625;0.57955185806468445530725830394658260047435760498046875;-2.335715701038534319877726375125348567962646484375;-0.1892873599881935986477543565342784859240055084228515625]
      mask Display: e = 0.06;c1 = [120 150 230]/255;c2 = ([120 150 230]+0)/383;c3 = ([120 150 230]+128)/383;patch([0 1 1 0],[0 0 1 1],c1);patch([0 1 1 1-e 1-e 0+e],[0 0 1 1-e 0+e 0+e],c2);patch([0 0 1 1-e 0+e 0+e],[0 1 1 1-e 1-e 0+e],c3);plot([0 1 1 0 0],[0 0 1 1 0]);disp('Weights');
  "IW{1,1}(150,:)'" : Constant  Value=[-2.371878147957687144042893123696558177471160888671875;0.0655044238850235049920200935957836918532848358154296875;1.0935592820533523994441793547593988478183746337890625;-1.664281943452273981876032848958857357501983642578125;-1.1107501073379155709375254446058534085750579833984375;0.86158354777594248208316685122554190456867218017578125]
      mask Display: e = 0.06;c1 = [120 150 230]/255;c2 = ([120 150 230]+0)/383;c3 = ([120 150 230]+128)/383;patch([0 1 1 0],[0 0 1 1],c1);patch([0 1 1 1-e 1-e 0+e],[0 0 1 1-e 0+e 0+e],c2);patch([0 0 1 1-e 0+e 0+e],[0 1 1 1-e 1-e 0+e],c3);plot([0 1 1 0 0],[0 0 1 1 0]);disp('Weights');
  "IW{1,1}(151,:)'" : Constant  Value=[1.195318942968249142921877137268893420696258544921875;-1.8334460053959091840880546442349441349506378173828125;0.1462588780386397668831222063090535812079906463623046875;-2.505645663401897760280689908540807664394378662109375;0.40232850050565016619685820842278189957141876220703125;0.43693649941245238377263149232021532952785491943359375]
      mask Display: e = 0.06;c1 = [120 150 230]/255;c2 = ([120 150 230]+0)/383;c3 = ([120 150 230]+128)/383;patch([0 1 1 0],[0 0 1 1],c1);patch([0 1 1 1-e 1-e 0+e],[0 0 1 1-e 0+e 0+e],c2);patch([0 0 1 1-e 0+e 0+e],[0 1 1 1-e 1-e 0+e],c3);plot([0 1 1 0 0],[0 0 1 1 0]);disp('Weights');
  "IW{1,1}(152,:)'" : Constant  Value=[1.74354932998822231837721119518391788005828857421875;1.0705548463252385626987006617127917706966400146484375;-0.70414634964965883145993075231672264635562896728515625;0.2078102812847431313247881234929081983864307403564453125;2.150747726622813882357831971603445708751678466796875;-1.5889491793305208222619739899528212845325469970703125]
      mask Display: e = 0.06;c1 = [120 150 230]/255;c2 = ([120 150 230]+0)/383;c3 = ([120 150 230]+128)/383;patch([0 1 1 0],[0 0 1 1],c1);patch([0 1 1 1-e 1-e 0+e],[0 0 1 1-e 0+e 0+e],c2);patch([0 0 1 1-e 0+e 0+e],[0 1 1 1-e 1-e 0+e],c3);plot([0 1 1 0 0],[0 0 1 1 0]);disp('Weights');
  "IW{1,1}(153,:)'" : Constant  Value=[1.90366393196154692901700400398112833499908447265625;0.2834736693426476161761229377589188516139984130859375;0.19353842037546475918219357481575571000576019287109375;0.8288521409726381516946958072367124259471893310546875;0.63140449741232196334550508254324086010456085205078125;-2.557226012769431289228805326274596154689788818359375]
      mask Display: e = 0.06;c1 = [120 150 230]/255;c2 = ([120 150 230]+0)/383;c3 = ([120 150 230]+128)/383;patch([0 1 1 0],[0 0 1 1],c1);patch([0 1 1 1-e 1-e 0+e],[0 0 1 1-e 0+e 0+e],c2);patch([0 0 1 1-e 0+e 0+e],[0 1 1 1-e 1-e 0+e],c3);plot([0 1 1 0 0],[0 0 1 1 0]);disp('Weights');
  "IW{1,1}(154,:)'" : Constant  Value=[1.9977276479975056844295977498404681682586669921875;1.7548951916726165389803782090893946588039398193359375;-0.82191519881507424383215720808948390185832977294921875;-0.70626412948527106383522777832695282995700836181640625;-1.7409803629414941639197422773577272891998291015625;0.014657775493403475686182702020232682116329669952392578125]
      mask Display: e = 0.06;c1 = [120 150 230]/255;c2 = ([120 150 230]+0)/383;c3 = ([120 150 230]+128)/383;patch([0 1 1 0],[0 0 1 1],c1);patch([0 1 1 1-e 1-e 0+e],[0 0 1 1-e 0+e 0+e],c2);patch([0 0 1 1-e 0+e 0+e],[0 1 1 1-e 1-e 0+e],c3);plot([0 1 1 0 0],[0 0 1 1 0]);disp('Weights');
  "IW{1,1}(155,:)'" : Constant  Value=[1.8995122857974358066002196210320107638835906982421875;1.5043736154819209449584604953997768461704254150390625;0.606161129636155759925486563588492572307586669921875;-1.5373536548326269812747568721533752977848052978515625;-1.591438178414662285575786881963722407817840576171875;0.06951624823206754844040489160761353559792041778564453125]
      mask Display: e = 0.06;c1 = [120 150 230]/255;c2 = ([120 150 230]+0)/383;c3 = ([120 150 230]+128)/383;patch([0 1 1 0],[0 0 1 1],c1);patch([0 1 1 1-e 1-e 0+e],[0 0 1 1-e 0+e 0+e],c2);patch([0 0 1 1-e 0+e 0+e],[0 1 1 1-e 1-e 0+e],c3);plot([0 1 1 0 0],[0 0 1 1 0]);disp('Weights');
  "IW{1,1}(156,:)'" : Constant  Value=[-1.432272400282839530660794480354525148868560791015625;0.7148856169267936433442400812054984271526336669921875;1.91126977572871936672527226619422435760498046875;-1.4156832976934021761650228654616512358188629150390625;-1.43152917145521740849289926700294017791748046875;1.172722304933671910731618481804616749286651611328125]
      mask Display: e = 0.06;c1 = [120 150 230]/255;c2 = ([120 150 230]+0)/383;c3 = ([120 150 230]+128)/383;patch([0 1 1 0],[0 0 1 1],c1);patch([0 1 1 1-e 1-e 0+e],[0 0 1 1-e 0+e 0+e],c2);patch([0 0 1 1-e 0+e 0+e],[0 1 1 1-e 1-e 0+e],c3);plot([0 1 1 0 0],[0 0 1 1 0]);disp('Weights');
  "IW{1,1}(157,:)'" : Constant  Value=[0.82514023174911221847338538282201625406742095947265625;0.757110900603036096612186156562529504299163818359375;0.65557760546125887213264604724827222526073455810546875;-2.323048736401905234316700443741865456104278564453125;1.61220011486059622285438308608718216419219970703125;1.3432756129062823902131640352308750152587890625]
      mask Display: e = 0.06;c1 = [120 150 230]/255;c2 = ([120 150 230]+0)/383;c3 = ([120 150 230]+128)/383;patch([0 1 1 0],[0 0 1 1],c1);patch([0 1 1 1-e 1-e 0+e],[0 0 1 1-e 0+e 0+e],c2);patch([0 0 1 1-e 0+e 0+e],[0 1 1 1-e 1-e 0+e],c3);plot([0 1 1 0 0],[0 0 1 1 0]);disp('Weights');
  "IW{1,1}(158,:)'" : Constant  Value=[0.38374726574355821906436858625966124236583709716796875;2.428868757170236758469172855257056653499603271484375;0.54408138779493808723231040858081541955471038818359375;-1.23259760738301427096530460403300821781158447265625;-1.0722200840054967319048273566295392811298370361328125;-1.586090176180915189974029999575577676296234130859375]
      mask Display: e = 0.06;c1 = [120 150 230]/255;c2 = ([120 150 230]+0)/383;c3 = ([120 150 230]+128)/383;patch([0 1 1 0],[0 0 1 1],c1);patch([0 1 1 1-e 1-e 0+e],[0 0 1 1-e 0+e 0+e],c2);patch([0 0 1 1-e 0+e 0+e],[0 1 1 1-e 1-e 0+e],c3);plot([0 1 1 0 0],[0 0 1 1 0]);disp('Weights');
  "IW{1,1}(159,:)'" : Constant  Value=[-0.7914305279780506907627568580210208892822265625;0.47132121317842023966449005456524901092052459716796875;1.44208858715752352708250327850691974163055419921875;0.476617860247140645579833062583929859101772308349609375;-2.619735993718328881385559725458733737468719482421875;-1.1950057997358201067328309363801963627338409423828125]
      mask Display: e = 0.06;c1 = [120 150 230]/255;c2 = ([120 150 230]+0)/383;c3 = ([120 150 230]+128)/383;patch([0 1 1 0],[0 0 1 1],c1);patch([0 1 1 1-e 1-e 0+e],[0 0 1 1-e 0+e 0+e],c2);patch([0 0 1 1-e 0+e 0+e],[0 1 1 1-e 1-e 0+e],c3);plot([0 1 1 0 0],[0 0 1 1 0]);disp('Weights');
  "IW{1,1}(16,:)'" : Constant  Value=[-2.182584653355827075671413695090450346469879150390625;0.53292843233945574876742057313094846904277801513671875;-0.7324047339933541511669545798213221132755279541015625;1.2989992312042513145087241355213336646556854248046875;1.8509114306297467233974884948111139237880706787109375;0.84096746626827989512520389325800351798534393310546875]
      mask Display: e = 0.06;c1 = [120 150 230]/255;c2 = ([120 150 230]+0)/383;c3 = ([120 150 230]+128)/383;patch([0 1 1 0],[0 0 1 1],c1);patch([0 1 1 1-e 1-e 0+e],[0 0 1 1-e 0+e 0+e],c2);patch([0 0 1 1-e 0+e 0+e],[0 1 1 1-e 1-e 0+e],c3);plot([0 1 1 0 0],[0 0 1 1 0]);disp('Weights');
  "IW{1,1}(160,:)'" : Constant  Value=[0.1992861304654575393957571805003681220114231109619140625;-0.12307620847451239409764411902870051562786102294921875;0.52620993961508777392310776122030802071094512939453125;-0.7733096234141978442266918136738240718841552734375;2.730408771552901736612284366856329143047332763671875;-1.70247180339769510482028636033646762371063232421875]
      mask Display: e = 0.06;c1 = [120 150 230]/255;c2 = ([120 150 230]+0)/383;c3 = ([120 150 230]+128)/383;patch([0 1 1 0],[0 0 1 1],c1);patch([0 1 1 1-e 1-e 0+e],[0 0 1 1-e 0+e 0+e],c2);patch([0 0 1 1-e 0+e 0+e],[0 1 1 1-e 1-e 0+e],c3);plot([0 1 1 0 0],[0 0 1 1 0]);disp('Weights');
  "IW{1,1}(161,:)'" : Constant  Value=[1.2561145465200826976115422439761459827423095703125;0.7536662954489461441198727698065340518951416015625;1.69713449376881353458657031296752393245697021484375;-1.6434524699531518621142822667025029659271240234375;-1.6044760405030047412111571247805841267108917236328125;1.163716630696929765775848863995634019374847412109375]
      mask Display: e = 0.06;c1 = [120 150 230]/255;c2 = ([120 150 230]+0)/383;c3 = ([120 150 230]+128)/383;patch([0 1 1 0],[0 0 1 1],c1);patch([0 1 1 1-e 1-e 0+e],[0 0 1 1-e 0+e 0+e],c2);patch([0 0 1 1-e 0+e 0+e],[0 1 1 1-e 1-e 0+e],c3);plot([0 1 1 0 0],[0 0 1 1 0]);disp('Weights');
  "IW{1,1}(162,:)'" : Constant  Value=[-1.393618397515708817735458069364540278911590576171875;1.7802812511310273091424960512085817754268646240234375;0.67988738083755162477928024600259959697723388671875;-0.7051085406843842218194140514242462813854217529296875;1.7997269094511076925613224375410936772823333740234375;-1.4560033155896341394708315419848076999187469482421875]
      mask Display: e = 0.06;c1 = [120 150 230]/255;c2 = ([120 150 230]+0)/383;c3 = ([120 150 230]+128)/383;patch([0 1 1 0],[0 0 1 1],c1);patch([0 1 1 1-e 1-e 0+e],[0 0 1 1-e 0+e 0+e],c2);patch([0 0 1 1-e 0+e 0+e],[0 1 1 1-e 1-e 0+e],c3);plot([0 1 1 0 0],[0 0 1 1 0]);disp('Weights');
  "IW{1,1}(163,:)'" : Constant  Value=[2.36690799940245266697047554771415889263153076171875;-1.8830082419537854665492204730981029570102691650390625;-1.25677372203648918258522826363332569599151611328125;0.56294322916407402157545902809943072497844696044921875;0.44223548819071056836804700651555322110652923583984375;0.2315730932366526773069637101798434741795063018798828125]
      mask Display: e = 0.06;c1 = [120 150 230]/255;c2 = ([120 150 230]+0)/383;c3 = ([120 150 230]+128)/383;patch([0 1 1 0],[0 0 1 1],c1);patch([0 1 1 1-e 1-e 0+e],[0 0 1 1-e 0+e 0+e],c2);patch([0 0 1 1-e 0+e 0+e],[0 1 1 1-e 1-e 0+e],c3);plot([0 1 1 0 0],[0 0 1 1 0]);disp('Weights');
  "IW{1,1}(164,:)'" : Constant  Value=[0.62227996745830249647468690454843454062938690185546875;-1.757715537463049759736577470903284847736358642578125;-1.634668506778918395383470851811580359935760498046875;1.9413361169953484708372570821666158735752105712890625;0.0175177616589151895210019205251228413544595241546630859375;-1.2101222891833287587104450722108595073223114013671875]
      mask Display: e = 0.06;c1 = [120 150 230]/255;c2 = ([120 150 230]+0)/383;c3 = ([120 150 230]+128)/383;patch([0 1 1 0],[0 0 1 1],c1);patch([0 1 1 1-e 1-e 0+e],[0 0 1 1-e 0+e 0+e],c2);patch([0 0 1 1-e 0+e 0+e],[0 1 1 1-e 1-e 0+e],c3);plot([0 1 1 0 0],[0 0 1 1 0]);disp('Weights');
  "IW{1,1}(165,:)'" : Constant  Value=[0.1928854935379941959450178501356276683509349822998046875;1.6690556049158520313113740485277958214282989501953125;1.5230442642565533706289215842843987047672271728515625;1.9745224963000733708895495510660111904144287109375;-1.4326377401043546289116648040362633764743804931640625;0.63842207313354892850298938355990685522556304931640625]
      mask Display: e = 0.06;c1 = [120 150 230]/255;c2 = ([120 150 230]+0)/383;c3 = ([120 150 230]+128)/383;patch([0 1 1 0],[0 0 1 1],c1);patch([0 1 1 1-e 1-e 0+e],[0 0 1 1-e 0+e 0+e],c2);patch([0 0 1 1-e 0+e 0+e],[0 1 1 1-e 1-e 0+e],c3);plot([0 1 1 0 0],[0 0 1 1 0]);disp('Weights');
  "IW{1,1}(166,:)'" : Constant  Value=[-0.1411944164048974659220192506836610846221446990966796875;1.201565820266788708892136128270067274570465087890625;-1.8134476254245299742251518182456493377685546875;-1.676547451317807801984827165142633020877838134765625;-1.563853975439573940064974522101692855358123779296875;1.103561461826986001000250325887463986873626708984375]
      mask Display: e = 0.06;c1 = [120 150 230]/255;c2 = ([120 150 230]+0)/383;c3 = ([120 150 230]+128)/383;patch([0 1 1 0],[0 0 1 1],c1);patch([0 1 1 1-e 1-e 0+e],[0 0 1 1-e 0+e 0+e],c2);patch([0 0 1 1-e 0+e 0+e],[0 1 1 1-e 1-e 0+e],c3);plot([0 1 1 0 0],[0 0 1 1 0]);disp('Weights');
  "IW{1,1}(167,:)'" : Constant  Value=[0.75269520738986261942926603296655230224132537841796875;1.1262079189036577897553570437594316899776458740234375;-0.65730306605700750122167619338142685592174530029296875;-1.65447602312714092676060317899100482463836669921875;-0.0273490524187832428903988102319999597966670989990234375;2.520700592372717263600634396425448358058929443359375]
      mask Display: e = 0.06;c1 = [120 150 230]/255;c2 = ([120 150 230]+0)/383;c3 = ([120 150 230]+128)/383;patch([0 1 1 0],[0 0 1 1],c1);patch([0 1 1 1-e 1-e 0+e],[0 0 1 1-e 0+e 0+e],c2);patch([0 0 1 1-e 0+e 0+e],[0 1 1 1-e 1-e 0+e],c3);plot([0 1 1 0 0],[0 0 1 1 0]);disp('Weights');
  "IW{1,1}(168,:)'" : Constant  Value=[-0.9468719033487016378813905248534865677356719970703125;-1.6199594839439022120330946563626639544963836669921875;0.2993634720297759788110170120489783585071563720703125;-1.270578283199505609246671156142838299274444580078125;1.8675791265483587810791732408688403666019439697265625;1.63003008598706689014079529442824423313140869140625]
      mask Display: e = 0.06;c1 = [120 150 230]/255;c2 = ([120 150 230]+0)/383;c3 = ([120 150 230]+128)/383;patch([0 1 1 0],[0 0 1 1],c1);patch([0 1 1 1-e 1-e 0+e],[0 0 1 1-e 0+e 0+e],c2);patch([0 0 1 1-e 0+e 0+e],[0 1 1 1-e 1-e 0+e],c3);plot([0 1 1 0 0],[0 0 1 1 0]);disp('Weights');
  "IW{1,1}(169,:)'" : Constant  Value=[1.5973275488636142771525783246033824980258941650390625;-1.9356211642697902508558627232559956610202789306640625;-0.10188452885504746536771136788956937380135059356689453125;1.4081339192351816080872595193795859813690185546875;-1.8134257570415803773045126945362426340579986572265625;-0.48851152481033410790445259408443234860897064208984375]
      mask Display: e = 0.06;c1 = [120 150 230]/255;c2 = ([120 150 230]+0)/383;c3 = ([120 150 230]+128)/383;patch([0 1 1 0],[0 0 1 1],c1);patch([0 1 1 1-e 1-e 0+e],[0 0 1 1-e 0+e 0+e],c2);patch([0 0 1 1-e 0+e 0+e],[0 1 1 1-e 1-e 0+e],c3);plot([0 1 1 0 0],[0 0 1 1 0]);disp('Weights');
  "IW{1,1}(17,:)'" : Constant  Value=[0.684960840193479025828082740190438926219940185546875;0.251206845311593152114681970488163642585277557373046875;0.8343200766052716321752313888282515108585357666015625;-2.156031196037737185378091453458182513713836669921875;-0.10328224232981271513143184392902185209095478057861328125;2.357535747078573162838210919289849698543548583984375]
      mask Display: e = 0.06;c1 = [120 150 230]/255;c2 = ([120 150 230]+0)/383;c3 = ([120 150 230]+128)/383;patch([0 1 1 0],[0 0 1 1],c1);patch([0 1 1 1-e 1-e 0+e],[0 0 1 1-e 0+e 0+e],c2);patch([0 0 1 1-e 0+e 0+e],[0 1 1 1-e 1-e 0+e],c3);plot([0 1 1 0 0],[0 0 1 1 0]);disp('Weights');
  "IW{1,1}(170,:)'" : Constant  Value=[-0.82843820683536950610914573189802467823028564453125;-1.94766829896245230457907382515259087085723876953125;0.0732145520693616713714391153189353644847869873046875;2.315749328589705502423612415441311895847320556640625;0.963062832742960228671336153638549149036407470703125;0.7078333976440458474854722226154990494251251220703125]
      mask Display: e = 0.06;c1 = [120 150 230]/255;c2 = ([120 150 230]+0)/383;c3 = ([120 150 230]+128)/383;patch([0 1 1 0],[0 0 1 1],c1);patch([0 1 1 1-e 1-e 0+e],[0 0 1 1-e 0+e 0+e],c2);patch([0 0 1 1-e 0+e 0+e],[0 1 1 1-e 1-e 0+e],c3);plot([0 1 1 0 0],[0 0 1 1 0]);disp('Weights');
  "IW{1,1}(171,:)'" : Constant  Value=[-0.6834289419179249147617838389123789966106414794921875;1.12087105458314084671656019054353237152099609375;-0.113288319318506081057051915195188485085964202880859375;-2.146361814923336108762441654107533395290374755859375;-1.5933715678854578623457882713410072028636932373046875;-1.6769757498277935159336493597947992384433746337890625]
      mask Display: e = 0.06;c1 = [120 150 230]/255;c2 = ([120 150 230]+0)/383;c3 = ([120 150 230]+128)/383;patch([0 1 1 0],[0 0 1 1],c1);patch([0 1 1 1-e 1-e 0+e],[0 0 1 1-e 0+e 0+e],c2);patch([0 0 1 1-e 0+e 0+e],[0 1 1 1-e 1-e 0+e],c3);plot([0 1 1 0 0],[0 0 1 1 0]);disp('Weights');
  "IW{1,1}(172,:)'" : Constant  Value=[1.43015165356292417442318765097297728061676025390625;-1.0309919892614320957591189653612673282623291015625;1.2816109701559010858318288228474557399749755859375;-0.1539136066865478269516387399562518112361431121826171875;1.0183840511947710449902615437167696654796600341796875;-2.26929797751718265175213673501275479793548583984375]
      mask Display: e = 0.06;c1 = [120 150 230]/255;c2 = ([120 150 230]+0)/383;c3 = ([120 150 230]+128)/383;patch([0 1 1 0],[0 0 1 1],c1);patch([0 1 1 1-e 1-e 0+e],[0 0 1 1-e 0+e 0+e],c2);patch([0 0 1 1-e 0+e 0+e],[0 1 1 1-e 1-e 0+e],c3);plot([0 1 1 0 0],[0 0 1 1 0]);disp('Weights');
  "IW{1,1}(173,:)'" : Constant  Value=[-2.203419941589160213624154494027607142925262451171875;1.395040607831375734093626306275837123394012451171875;1.426808308001375369400420822785235941410064697265625;-0.139630807195123385344714961320278234779834747314453125;-0.26779070968029905497331810693140141665935516357421875;1.589763474757238004286818977561779320240020751953125]
      mask Display: e = 0.06;c1 = [120 150 230]/255;c2 = ([120 150 230]+0)/383;c3 = ([120 150 230]+128)/383;patch([0 1 1 0],[0 0 1 1],c1);patch([0 1 1 1-e 1-e 0+e],[0 0 1 1-e 0+e 0+e],c2);patch([0 0 1 1-e 0+e 0+e],[0 1 1 1-e 1-e 0+e],c3);plot([0 1 1 0 0],[0 0 1 1 0]);disp('Weights');
  "IW{1,1}(174,:)'" : Constant  Value=[-1.43331558299876871132028099964372813701629638671875;1.179608273437757315349472264642827212810516357421875;1.8494310349715039620832612854428589344024658203125;-1.3984713490584879114209115869016386568546295166015625;0.07855224157102190518653372919288813136518001556396484375;1.576933852426430693327574772411026060581207275390625]
      mask Display: e = 0.06;c1 = [120 150 230]/255;c2 = ([120 150 230]+0)/383;c3 = ([120 150 230]+128)/383;patch([0 1 1 0],[0 0 1 1],c1);patch([0 1 1 1-e 1-e 0+e],[0 0 1 1-e 0+e 0+e],c2);patch([0 0 1 1-e 0+e 0+e],[0 1 1 1-e 1-e 0+e],c3);plot([0 1 1 0 0],[0 0 1 1 0]);disp('Weights');
  "IW{1,1}(175,:)'" : Constant  Value=[0.362779543529922976485835306448279879987239837646484375;0.5953092400438293463338368383119814097881317138671875;2.84324475068556381529560894705355167388916015625;-0.72419810337774592756687752626021392643451690673828125;1.8584016606515267877597352708107791841030120849609375;-0.74015514996215614473840105347335338592529296875]
      mask Display: e = 0.06;c1 = [120 150 230]/255;c2 = ([120 150 230]+0)/383;c3 = ([120 150 230]+128)/383;patch([0 1 1 0],[0 0 1 1],c1);patch([0 1 1 1-e 1-e 0+e],[0 0 1 1-e 0+e 0+e],c2);patch([0 0 1 1-e 0+e 0+e],[0 1 1 1-e 1-e 0+e],c3);plot([0 1 1 0 0],[0 0 1 1 0]);disp('Weights');
  "IW{1,1}(176,:)'" : Constant  Value=[-1.913541267317007577020149255986325442790985107421875;0.1760749918515901735194262300865375436842441558837890625;-0.321934797882384049483306398542481474578380584716796875;0.13350091766338090248922298997058533132076263427734375;-1.960620306631197795610432876856066286563873291015625;-1.636734200102921921171628127922303974628448486328125]
      mask Display: e = 0.06;c1 = [120 150 230]/255;c2 = ([120 150 230]+0)/383;c3 = ([120 150 230]+128)/383;patch([0 1 1 0],[0 0 1 1],c1);patch([0 1 1 1-e 1-e 0+e],[0 0 1 1-e 0+e 0+e],c2);patch([0 0 1 1-e 0+e 0+e],[0 1 1 1-e 1-e 0+e],c3);plot([0 1 1 0 0],[0 0 1 1 0]);disp('Weights');
  "IW{1,1}(177,:)'" : Constant  Value=[0.10914363231892930394817398109807982109487056732177734375;1.2421993411997294121107415776350535452365875244140625;-1.775866619294888426594525299151428043842315673828125;1.4534976222479991658786957486881874501705169677734375;1.3161899387097271141300325325573794543743133544921875;-1.788032973073453657519849002710543572902679443359375]
      mask Display: e = 0.06;c1 = [120 150 230]/255;c2 = ([120 150 230]+0)/383;c3 = ([120 150 230]+128)/383;patch([0 1 1 0],[0 0 1 1],c1);patch([0 1 1 1-e 1-e 0+e],[0 0 1 1-e 0+e 0+e],c2);patch([0 0 1 1-e 0+e 0+e],[0 1 1 1-e 1-e 0+e],c3);plot([0 1 1 0 0],[0 0 1 1 0]);disp('Weights');
  "IW{1,1}(178,:)'" : Constant  Value=[0.251832131382804080832471527173765935003757476806640625;-0.2618183252561914198253134600236080586910247802734375;2.17605497428670080495294314459897577762603759765625;0.78172102422489098128011164590134285390377044677734375;-0.5649339081922690741777159928460605442523956298828125;-2.26733576628458077806271830922923982143402099609375]
      mask Display: e = 0.06;c1 = [120 150 230]/255;c2 = ([120 150 230]+0)/383;c3 = ([120 150 230]+128)/383;patch([0 1 1 0],[0 0 1 1],c1);patch([0 1 1 1-e 1-e 0+e],[0 0 1 1-e 0+e 0+e],c2);patch([0 0 1 1-e 0+e 0+e],[0 1 1 1-e 1-e 0+e],c3);plot([0 1 1 0 0],[0 0 1 1 0]);disp('Weights');
  "IW{1,1}(179,:)'" : Constant  Value=[-0.9141232682898705608209866113611496984958648681640625;-1.195415460660665285530512846889905631542205810546875;-1.1276860838539028986104995055939070880413055419921875;-1.903941239729394663271477838861756026744842529296875;-1.4392263604690793687979066817206330597400665283203125;1.514434581966808135433666393510065972805023193359375]
      mask Display: e = 0.06;c1 = [120 150 230]/255;c2 = ([120 150 230]+0)/383;c3 = ([120 150 230]+128)/383;patch([0 1 1 0],[0 0 1 1],c1);patch([0 1 1 1-e 1-e 0+e],[0 0 1 1-e 0+e 0+e],c2);patch([0 0 1 1-e 0+e 0+e],[0 1 1 1-e 1-e 0+e],c3);plot([0 1 1 0 0],[0 0 1 1 0]);disp('Weights');
  "IW{1,1}(18,:)'" : Constant  Value=[-0.463539690701430806551996965936268679797649383544921875;-1.0827868239643156922369371386594139039516448974609375;-0.2328899790603215780304680038170772604644298553466796875;-1.3653160291580845875358818375389091670513153076171875;1.740641620431479186237311296281404793262481689453125;-2.351137964263084523253155566635541617870330810546875]
      mask Display: e = 0.06;c1 = [120 150 230]/255;c2 = ([120 150 230]+0)/383;c3 = ([120 150 230]+128)/383;patch([0 1 1 0],[0 0 1 1],c1);patch([0 1 1 1-e 1-e 0+e],[0 0 1 1-e 0+e 0+e],c2);patch([0 0 1 1-e 0+e 0+e],[0 1 1 1-e 1-e 0+e],c3);plot([0 1 1 0 0],[0 0 1 1 0]);disp('Weights');
  "IW{1,1}(180,:)'" : Constant  Value=[0.377600316523597545614876480613020248711109161376953125;-2.090982565807624649067975042271427810192108154296875;1.98927613224057520113774444325827062129974365234375;-1.5685309078383842251724900052067823708057403564453125;0.70690708108590183389452477058512158691883087158203125;-0.30579156243345717580695009019109420478343963623046875]
      mask Display: e = 0.06;c1 = [120 150 230]/255;c2 = ([120 150 230]+0)/383;c3 = ([120 150 230]+128)/383;patch([0 1 1 0],[0 0 1 1],c1);patch([0 1 1 1-e 1-e 0+e],[0 0 1 1-e 0+e 0+e],c2);patch([0 0 1 1-e 0+e 0+e],[0 1 1 1-e 1-e 0+e],c3);plot([0 1 1 0 0],[0 0 1 1 0]);disp('Weights');
  "IW{1,1}(181,:)'" : Constant  Value=[-1.2290816987278170291375545275514014065265655517578125;1.9792271299083861180179155780933797359466552734375;2.03884379012881655768296695896424353122711181640625;0.63970092355328345146148194544366560876369476318359375;-1.0639003614239681549946681116125546395778656005859375;-0.42299687873168301255333290100679732859134674072265625]
      mask Display: e = 0.06;c1 = [120 150 230]/255;c2 = ([120 150 230]+0)/383;c3 = ([120 150 230]+128)/383;patch([0 1 1 0],[0 0 1 1],c1);patch([0 1 1 1-e 1-e 0+e],[0 0 1 1-e 0+e 0+e],c2);patch([0 0 1 1-e 0+e 0+e],[0 1 1 1-e 1-e 0+e],c3);plot([0 1 1 0 0],[0 0 1 1 0]);disp('Weights');
  "IW{1,1}(182,:)'" : Constant  Value=[-2.41075024436140683548046581563539803028106689453125;1.715023148449488221700676149339415132999420166015625;-1.173661308180590001626342200324870645999908447265625;-0.83873926834681877817700978994253091514110565185546875;-0.86319966629758637655100983465672470629215240478515625;0.369731954637447735034783136143232695758342742919921875]
      mask Display: e = 0.06;c1 = [120 150 230]/255;c2 = ([120 150 230]+0)/383;c3 = ([120 150 230]+128)/383;patch([0 1 1 0],[0 0 1 1],c1);patch([0 1 1 1-e 1-e 0+e],[0 0 1 1-e 0+e 0+e],c2);patch([0 0 1 1-e 0+e 0+e],[0 1 1 1-e 1-e 0+e],c3);plot([0 1 1 0 0],[0 0 1 1 0]);disp('Weights');
  "IW{1,1}(183,:)'" : Constant  Value=[0.24003323824219513493716249286080710589885711669921875;-0.57964512078611374334968786570243537425994873046875;-2.407706178026854271223555770120583474636077880859375;-1.8891159331541260701925466491957195103168487548828125;-0.5027379684860040498506350559182465076446533203125;1.356225039940706533769798625144176185131072998046875]
      mask Display: e = 0.06;c1 = [120 150 230]/255;c2 = ([120 150 230]+0)/383;c3 = ([120 150 230]+128)/383;patch([0 1 1 0],[0 0 1 1],c1);patch([0 1 1 1-e 1-e 0+e],[0 0 1 1-e 0+e 0+e],c2);patch([0 0 1 1-e 0+e 0+e],[0 1 1 1-e 1-e 0+e],c3);plot([0 1 1 0 0],[0 0 1 1 0]);disp('Weights');
  "IW{1,1}(184,:)'" : Constant  Value=[-0.3750699757125752764608250799938105046749114990234375;0.713073730094456958994442175026051700115203857421875;0.9391126042123134620709379305480979382991790771484375;2.507566608735882329739297347259707748889923095703125;2.044777395777696682444002362899482250213623046875;0.326268739096983340086666203205822966992855072021484375]
      mask Display: e = 0.06;c1 = [120 150 230]/255;c2 = ([120 150 230]+0)/383;c3 = ([120 150 230]+128)/383;patch([0 1 1 0],[0 0 1 1],c1);patch([0 1 1 1-e 1-e 0+e],[0 0 1 1-e 0+e 0+e],c2);patch([0 0 1 1-e 0+e 0+e],[0 1 1 1-e 1-e 0+e],c3);plot([0 1 1 0 0],[0 0 1 1 0]);disp('Weights');
  "IW{1,1}(185,:)'" : Constant  Value=[1.81991160492575598794928737333975732326507568359375;-1.8366390655517417229702914482913911342620849609375;1.538888213768264900949134244001470506191253662109375;-0.74502651205524317301609471542178653180599212646484375;1.21442122944598995815113084972836077213287353515625;-0.75906986615740834611898435468901880085468292236328125]
      mask Display: e = 0.06;c1 = [120 150 230]/255;c2 = ([120 150 230]+0)/383;c3 = ([120 150 230]+128)/383;patch([0 1 1 0],[0 0 1 1],c1);patch([0 1 1 1-e 1-e 0+e],[0 0 1 1-e 0+e 0+e],c2);patch([0 0 1 1-e 0+e 0+e],[0 1 1 1-e 1-e 0+e],c3);plot([0 1 1 0 0],[0 0 1 1 0]);disp('Weights');
  "IW{1,1}(186,:)'" : Constant  Value=[-1.76042009889694828217443500761874020099639892578125;-1.32252744832659718809964033425785601139068603515625;1.643670858772816156800899989320896565914154052734375;1.406641601085273141080733694252558052539825439453125;-1.5564026576936915713389453230774961411952972412109375;-0.6019901660603128590310006984509527683258056640625]
      mask Display: e = 0.06;c1 = [120 150 230]/255;c2 = ([120 150 230]+0)/383;c3 = ([120 150 230]+128)/383;patch([0 1 1 0],[0 0 1 1],c1);patch([0 1 1 1-e 1-e 0+e],[0 0 1 1-e 0+e 0+e],c2);patch([0 0 1 1-e 0+e 0+e],[0 1 1 1-e 1-e 0+e],c3);plot([0 1 1 0 0],[0 0 1 1 0]);disp('Weights');
  "IW{1,1}(187,:)'" : Constant  Value=[-1.5003614435489238676524337279261089861392974853515625;-1.79274679226861355374467166257090866565704345703125;0.26686417285017982603534392183064483106136322021484375;-0.8990800927070361492354777510627172887325286865234375;1.201390717500816496254856247105635702610015869140625;1.98504798949270622188123525120317935943603515625]
      mask Display: e = 0.06;c1 = [120 150 230]/255;c2 = ([120 150 230]+0)/383;c3 = ([120 150 230]+128)/383;patch([0 1 1 0],[0 0 1 1],c1);patch([0 1 1 1-e 1-e 0+e],[0 0 1 1-e 0+e 0+e],c2);patch([0 0 1 1-e 0+e 0+e],[0 1 1 1-e 1-e 0+e],c3);plot([0 1 1 0 0],[0 0 1 1 0]);disp('Weights');
  "IW{1,1}(188,:)'" : Constant  Value=[-2.15903796536142156270443592802621424198150634765625;2.037782307147949278913756643305532634258270263671875;0.66972246691830650267007740694680251181125640869140625;0.85911052001335785899271968446555547416210174560546875;0.126425933822923830529560973445768468081951141357421875;-1.0821348361794835835070216489839367568492889404296875]
      mask Display: e = 0.06;c1 = [120 150 230]/255;c2 = ([120 150 230]+0)/383;c3 = ([120 150 230]+128)/383;patch([0 1 1 0],[0 0 1 1],c1);patch([0 1 1 1-e 1-e 0+e],[0 0 1 1-e 0+e 0+e],c2);patch([0 0 1 1-e 0+e 0+e],[0 1 1 1-e 1-e 0+e],c3);plot([0 1 1 0 0],[0 0 1 1 0]);disp('Weights');
  "IW{1,1}(189,:)'" : Constant  Value=[0.469085805087207152741513027649489231407642364501953125;0.90765500750866190404764211052679456770420074462890625;-1.9473825614531194982959050321369431912899017333984375;0.74180298087968876696862707831314764916896820068359375;1.8450146148153498959487706088111735880374908447265625;1.316028597631177632365506724454462528228759765625]
      mask Display: e = 0.06;c1 = [120 150 230]/255;c2 = ([120 150 230]+0)/383;c3 = ([120 150 230]+128)/383;patch([0 1 1 0],[0 0 1 1],c1);patch([0 1 1 1-e 1-e 0+e],[0 0 1 1-e 0+e 0+e],c2);patch([0 0 1 1-e 0+e 0+e],[0 1 1 1-e 1-e 0+e],c3);plot([0 1 1 0 0],[0 0 1 1 0]);disp('Weights');
  "IW{1,1}(19,:)'" : Constant  Value=[-1.10438004489299590460404942859895527362823486328125;0.304688298402403578979402709592250175774097442626953125;-2.1356466160969720391449300223030149936676025390625;1.91542929194283839677837022463791072368621826171875;1.3679202226428890387666115202591754496097564697265625;-0.53929786985294725365491785851190797984600067138671875]
      mask Display: e = 0.06;c1 = [120 150 230]/255;c2 = ([120 150 230]+0)/383;c3 = ([120 150 230]+128)/383;patch([0 1 1 0],[0 0 1 1],c1);patch([0 1 1 1-e 1-e 0+e],[0 0 1 1-e 0+e 0+e],c2);patch([0 0 1 1-e 0+e 0+e],[0 1 1 1-e 1-e 0+e],c3);plot([0 1 1 0 0],[0 0 1 1 0]);disp('Weights');
  "IW{1,1}(190,:)'" : Constant  Value=[-2.798613352490973316122335745603777468204498291015625;-0.89039250390928004197377276796032674610614776611328125;-0.12162071479979406907201422427533543668687343597412109375;0.25126132918326515852669444939238019287586212158203125;-1.3190856224946825303590003386489115655422210693359375;-0.868641969301002792036570099298842251300811767578125]
      mask Display: e = 0.06;c1 = [120 150 230]/255;c2 = ([120 150 230]+0)/383;c3 = ([120 150 230]+128)/383;patch([0 1 1 0],[0 0 1 1],c1);patch([0 1 1 1-e 1-e 0+e],[0 0 1 1-e 0+e 0+e],c2);patch([0 0 1 1-e 0+e 0+e],[0 1 1 1-e 1-e 0+e],c3);plot([0 1 1 0 0],[0 0 1 1 0]);disp('Weights');
  "IW{1,1}(191,:)'" : Constant  Value=[-0.64701961684668163332645463015069253742694854736328125;-0.77079569765798694458425188713590614497661590576171875;0.7119663152272917017171494080685079097747802734375;1.8391199585669106841834263832424767315387725830078125;2.27357069974699843584176051081158220767974853515625;0.77739315001271702687546394372475333511829376220703125]
      mask Display: e = 0.06;c1 = [120 150 230]/255;c2 = ([120 150 230]+0)/383;c3 = ([120 150 230]+128)/383;patch([0 1 1 0],[0 0 1 1],c1);patch([0 1 1 1-e 1-e 0+e],[0 0 1 1-e 0+e 0+e],c2);patch([0 0 1 1-e 0+e 0+e],[0 1 1 1-e 1-e 0+e],c3);plot([0 1 1 0 0],[0 0 1 1 0]);disp('Weights');
  "IW{1,1}(192,:)'" : Constant  Value=[-0.10696397557975302616828372492818743921816349029541015625;-2.401178223514067067156929624616168439388275146484375;-0.7192323135945144496616876494954340159893035888671875;0.420091135851151875613140873610973358154296875;0.04943986885218358551252748611659626476466655731201171875;2.436559506204262870454613221227191388607025146484375]
      mask Display: e = 0.06;c1 = [120 150 230]/255;c2 = ([120 150 230]+0)/383;c3 = ([120 150 230]+128)/383;patch([0 1 1 0],[0 0 1 1],c1);patch([0 1 1 1-e 1-e 0+e],[0 0 1 1-e 0+e 0+e],c2);patch([0 0 1 1-e 0+e 0+e],[0 1 1 1-e 1-e 0+e],c3);plot([0 1 1 0 0],[0 0 1 1 0]);disp('Weights');
  "IW{1,1}(193,:)'" : Constant  Value=[2.49023522255334039954277614015154540538787841796875;0.9766229313152672286690858527435921132564544677734375;0.3773360613760274873129674233496189117431640625;-0.3689153688349373627630711780511774122714996337890625;1.8220447467196916324638777950895018875598907470703125;1.0396339147525062163168740880792029201984405517578125]
      mask Display: e = 0.06;c1 = [120 150 230]/255;c2 = ([120 150 230]+0)/383;c3 = ([120 150 230]+128)/383;patch([0 1 1 0],[0 0 1 1],c1);patch([0 1 1 1-e 1-e 0+e],[0 0 1 1-e 0+e 0+e],c2);patch([0 0 1 1-e 0+e 0+e],[0 1 1 1-e 1-e 0+e],c3);plot([0 1 1 0 0],[0 0 1 1 0]);disp('Weights');
  "IW{1,1}(194,:)'" : Constant  Value=[0.97507596248076311429286988641251809895038604736328125;1.4899790810369053506434511291445232927799224853515625;-1.5404785438154353638395832604146562516689300537109375;-0.0813962354063614001997706282054423354566097259521484375;-2.400906972865758604029906564392149448394775390625;0.61260297842618671726455659154453314840793609619140625]
      mask Display: e = 0.06;c1 = [120 150 230]/255;c2 = ([120 150 230]+0)/383;c3 = ([120 150 230]+128)/383;patch([0 1 1 0],[0 0 1 1],c1);patch([0 1 1 1-e 1-e 0+e],[0 0 1 1-e 0+e 0+e],c2);patch([0 0 1 1-e 0+e 0+e],[0 1 1 1-e 1-e 0+e],c3);plot([0 1 1 0 0],[0 0 1 1 0]);disp('Weights');
  "IW{1,1}(195,:)'" : Constant  Value=[-0.981933763261455538895461359061300754547119140625;-1.663314354523703020305447353166528046131134033203125;-1.6478984126948532651368850565631873905658721923828125;1.4187285680284016375907185647520236670970916748046875;-0.86810457355834980130993017155560664832592010498046875;1.6054670250449312174367832994903437793254852294921875]
      mask Display: e = 0.06;c1 = [120 150 230]/255;c2 = ([120 150 230]+0)/383;c3 = ([120 150 230]+128)/383;patch([0 1 1 0],[0 0 1 1],c1);patch([0 1 1 1-e 1-e 0+e],[0 0 1 1-e 0+e 0+e],c2);patch([0 0 1 1-e 0+e 0+e],[0 1 1 1-e 1-e 0+e],c3);plot([0 1 1 0 0],[0 0 1 1 0]);disp('Weights');
  "IW{1,1}(196,:)'" : Constant  Value=[-0.355111011807442256138500624729203991591930389404296875;1.1923614645870592720910963180358521640300750732421875;0.408750903375600938005618445458821952342987060546875;-0.0437136169398301410726759286262677051126956939697265625;1.181699593369221812366731683141551911830902099609375;3.321956530624714520882889701169915497303009033203125]
      mask Display: e = 0.06;c1 = [120 150 230]/255;c2 = ([120 150 230]+0)/383;c3 = ([120 150 230]+128)/383;patch([0 1 1 0],[0 0 1 1],c1);patch([0 1 1 1-e 1-e 0+e],[0 0 1 1-e 0+e 0+e],c2);patch([0 0 1 1-e 0+e 0+e],[0 1 1 1-e 1-e 0+e],c3);plot([0 1 1 0 0],[0 0 1 1 0]);disp('Weights');
  "IW{1,1}(197,:)'" : Constant  Value=[1.26070496245477858821004701894707977771759033203125;-2.568044786703559179130706979776732623577117919921875;-0.872325938494356467600709947873838245868682861328125;-0.356324343898632267535475648401188664138317108154296875;-0.7216094350829045378503678875858895480632781982421875;1.3502792920849666646887499155127443373203277587890625]
      mask Display: e = 0.06;c1 = [120 150 230]/255;c2 = ([120 150 230]+0)/383;c3 = ([120 150 230]+128)/383;patch([0 1 1 0],[0 0 1 1],c1);patch([0 1 1 1-e 1-e 0+e],[0 0 1 1-e 0+e 0+e],c2);patch([0 0 1 1-e 0+e 0+e],[0 1 1 1-e 1-e 0+e],c3);plot([0 1 1 0 0],[0 0 1 1 0]);disp('Weights');
  "IW{1,1}(198,:)'" : Constant  Value=[-2.016815815094731068057853917707689106464385986328125;0.477702421989108838573656612425111234188079833984375;-1.9543240507141863560036654234863817691802978515625;0.6279029292680184948238775177742354571819305419921875;-0.11985751079179952915954032732770428992807865142822265625;1.5985978163717182720660048289573751389980316162109375]
      mask Display: e = 0.06;c1 = [120 150 230]/255;c2 = ([120 150 230]+0)/383;c3 = ([120 150 230]+128)/383;patch([0 1 1 0],[0 0 1 1],c1);patch([0 1 1 1-e 1-e 0+e],[0 0 1 1-e 0+e 0+e],c2);patch([0 0 1 1-e 0+e 0+e],[0 1 1 1-e 1-e 0+e],c3);plot([0 1 1 0 0],[0 0 1 1 0]);disp('Weights');
  "IW{1,1}(199,:)'" : Constant  Value=[1.6420216007108157096894274218357168138027191162109375;0.62292703541944438594413213650113902986049652099609375;-1.2750083454424625539758153536240570247173309326171875;-1.7615003170172374158397587962099350988864898681640625;-1.355108456066237199166835125652141869068145751953125;-1.285975679500478197070378882926888763904571533203125]
      mask Display: e = 0.06;c1 = [120 150 230]/255;c2 = ([120 150 230]+0)/383;c3 = ([120 150 230]+128)/383;patch([0 1 1 0],[0 0 1 1],c1);patch([0 1 1 1-e 1-e 0+e],[0 0 1 1-e 0+e 0+e],c2);patch([0 0 1 1-e 0+e 0+e],[0 1 1 1-e 1-e 0+e],c3);plot([0 1 1 0 0],[0 0 1 1 0]);disp('Weights');
  "IW{1,1}(2,:)'" : Constant  Value=[-0.4334872891652568061005013078101910650730133056640625;1.783798845788539200185596200753934681415557861328125;-1.7417208660352994087361366837285459041595458984375;-1.0154806558674229766126018148497678339481353759765625;1.0316487303343213621786844669259153306484222412109375;1.7290812864770668255687269265763461589813232421875]
      mask Display: e = 0.06;c1 = [120 150 230]/255;c2 = ([120 150 230]+0)/383;c3 = ([120 150 230]+128)/383;patch([0 1 1 0],[0 0 1 1],c1);patch([0 1 1 1-e 1-e 0+e],[0 0 1 1-e 0+e 0+e],c2);patch([0 0 1 1-e 0+e 0+e],[0 1 1 1-e 1-e 0+e],c3);plot([0 1 1 0 0],[0 0 1 1 0]);disp('Weights');
  "IW{1,1}(20,:)'" : Constant  Value=[-1.84814829199895225286809363751672208309173583984375;-1.950826713719362448529182074707932770252227783203125;-0.66466417417492607011553218399058096110820770263671875;0.74719943008052192023882298599346540868282318115234375;1.7665192837907202072500467693316750228404998779296875;0.33105239409209696876956741107278503477573394775390625]
      mask Display: e = 0.06;c1 = [120 150 230]/255;c2 = ([120 150 230]+0)/383;c3 = ([120 150 230]+128)/383;patch([0 1 1 0],[0 0 1 1],c1);patch([0 1 1 1-e 1-e 0+e],[0 0 1 1-e 0+e 0+e],c2);patch([0 0 1 1-e 0+e 0+e],[0 1 1 1-e 1-e 0+e],c3);plot([0 1 1 0 0],[0 0 1 1 0]);disp('Weights');
  "IW{1,1}(200,:)'" : Constant  Value=[1.7131816640219759140251198914484120905399322509765625;-1.3711589552054286311744135673507116734981536865234375;-0.1069080316925972440333936219758470542728900909423828125;-1.91415667953703039216861725435592234134674072265625;-1.066515339354911162672578939236700534820556640625;-1.2853445268178749216758660622872412204742431640625]
      mask Display: e = 0.06;c1 = [120 150 230]/255;c2 = ([120 150 230]+0)/383;c3 = ([120 150 230]+128)/383;patch([0 1 1 0],[0 0 1 1],c1);patch([0 1 1 1-e 1-e 0+e],[0 0 1 1-e 0+e 0+e],c2);patch([0 0 1 1-e 0+e 0+e],[0 1 1 1-e 1-e 0+e],c3);plot([0 1 1 0 0],[0 0 1 1 0]);disp('Weights');
  "IW{1,1}(21,:)'" : Constant  Value=[-0.1622876571547901269898517284673289395868778228759765625;-1.8232250315500964088499813442467711865901947021484375;1.6491138626872612338303270007600076496601104736328125;-1.082588801541390921556740067899227142333984375;-1.3103603765620646104395063957781530916690826416015625;1.5619835645533493018177750855102203786373138427734375]
      mask Display: e = 0.06;c1 = [120 150 230]/255;c2 = ([120 150 230]+0)/383;c3 = ([120 150 230]+128)/383;patch([0 1 1 0],[0 0 1 1],c1);patch([0 1 1 1-e 1-e 0+e],[0 0 1 1-e 0+e 0+e],c2);patch([0 0 1 1-e 0+e 0+e],[0 1 1 1-e 1-e 0+e],c3);plot([0 1 1 0 0],[0 0 1 1 0]);disp('Weights');
  "IW{1,1}(22,:)'" : Constant  Value=[0.55863196887118593547683076394605450332164764404296875;0.411792296457283935051663092963281087577342987060546875;-0.66256340928208790064246613837894983589649200439453125;0.4363614686136843001662555252551101148128509521484375;-2.8883958257383017809161174227483570575714111328125;-1.3099339874561051200174688347033224999904632568359375]
      mask Display: e = 0.06;c1 = [120 150 230]/255;c2 = ([120 150 230]+0)/383;c3 = ([120 150 230]+128)/383;patch([0 1 1 0],[0 0 1 1],c1);patch([0 1 1 1-e 1-e 0+e],[0 0 1 1-e 0+e 0+e],c2);patch([0 0 1 1-e 0+e 0+e],[0 1 1 1-e 1-e 0+e],c3);plot([0 1 1 0 0],[0 0 1 1 0]);disp('Weights');
  "IW{1,1}(23,:)'" : Constant  Value=[0.95056149418465085698670691272127442061901092529296875;1.7070414428342404189464787123142741620540618896484375;0.64485835583116213332033339611371047794818878173828125;-1.17252228181764106551554505131207406520843505859375;-2.5431878199653770167287802905775606632232666015625;-0.72171829564721978744756825108197517693042755126953125]
      mask Display: e = 0.06;c1 = [120 150 230]/255;c2 = ([120 150 230]+0)/383;c3 = ([120 150 230]+128)/383;patch([0 1 1 0],[0 0 1 1],c1);patch([0 1 1 1-e 1-e 0+e],[0 0 1 1-e 0+e 0+e],c2);patch([0 0 1 1-e 0+e 0+e],[0 1 1 1-e 1-e 0+e],c3);plot([0 1 1 0 0],[0 0 1 1 0]);disp('Weights');
  "IW{1,1}(24,:)'" : Constant  Value=[1.78507205727958062624338708701543509960174560546875;-1.166477066667431561342027634964324533939361572265625;-0.224974259441496460265597079342114739120006561279296875;-1.7905410185546630774666709839948453009128570556640625;1.675611541902392698233370538218878209590911865234375;-1.0554052852767303871672766035771928727626800537109375]
      mask Display: e = 0.06;c1 = [120 150 230]/255;c2 = ([120 150 230]+0)/383;c3 = ([120 150 230]+128)/383;patch([0 1 1 0],[0 0 1 1],c1);patch([0 1 1 1-e 1-e 0+e],[0 0 1 1-e 0+e 0+e],c2);patch([0 0 1 1-e 0+e 0+e],[0 1 1 1-e 1-e 0+e],c3);plot([0 1 1 0 0],[0 0 1 1 0]);disp('Weights');
  "IW{1,1}(25,:)'" : Constant  Value=[0.0507380014387421862664950822363607585430145263671875;-0.48762868314374940847955031131277792155742645263671875;1.0598989113691985597398570462246425449848175048828125;-1.728061228712839625387687192414887249469757080078125;1.27472502490148631437705262214876711368560791015625;-2.35756119525967022809709305875003337860107421875]
      mask Display: e = 0.06;c1 = [120 150 230]/255;c2 = ([120 150 230]+0)/383;c3 = ([120 150 230]+128)/383;patch([0 1 1 0],[0 0 1 1],c1);patch([0 1 1 1-e 1-e 0+e],[0 0 1 1-e 0+e 0+e],c2);patch([0 0 1 1-e 0+e 0+e],[0 1 1 1-e 1-e 0+e],c3);plot([0 1 1 0 0],[0 0 1 1 0]);disp('Weights');
  "IW{1,1}(26,:)'" : Constant  Value=[-0.61167514444733306344659240494365803897380828857421875;-1.4476690889416652385790484913741238415241241455078125;1.9338862734836610446365057214279659092426300048828125;-0.62702219583894958088166049492429010570049285888671875;1.6515382103993896389937390267732553184032440185546875;-1.62916016514775296997186160297133028507232666015625]
      mask Display: e = 0.06;c1 = [120 150 230]/255;c2 = ([120 150 230]+0)/383;c3 = ([120 150 230]+128)/383;patch([0 1 1 0],[0 0 1 1],c1);patch([0 1 1 1-e 1-e 0+e],[0 0 1 1-e 0+e 0+e],c2);patch([0 0 1 1-e 0+e 0+e],[0 1 1 1-e 1-e 0+e],c3);plot([0 1 1 0 0],[0 0 1 1 0]);disp('Weights');
  "IW{1,1}(27,:)'" : Constant  Value=[1.2555349287219590426190052312449552118778228759765625;0.9185929270396737678083809441886842250823974609375;1.2707542106650209223772662880946882069110870361328125;1.8851925145696901697789371610269881784915924072265625;-1.5906057215623869982579208226525224745273590087890625;-1.20734507129496737576346276910044252872467041015625]
      mask Display: e = 0.06;c1 = [120 150 230]/255;c2 = ([120 150 230]+0)/383;c3 = ([120 150 230]+128)/383;patch([0 1 1 0],[0 0 1 1],c1);patch([0 1 1 1-e 1-e 0+e],[0 0 1 1-e 0+e 0+e],c2);patch([0 0 1 1-e 0+e 0+e],[0 1 1 1-e 1-e 0+e],c3);plot([0 1 1 0 0],[0 0 1 1 0]);disp('Weights');
  "IW{1,1}(28,:)'" : Constant  Value=[-0.403484541198686763596725768366013653576374053955078125;-1.91806215914525779453470022417604923248291015625;-0.242860422457327640444191274582408368587493896484375;-1.6019839283553363173950856435112655162811279296875;1.253814074265096056848278749384917318820953369140625;-1.826022606039152673673697790945880115032196044921875]
      mask Display: e = 0.06;c1 = [120 150 230]/255;c2 = ([120 150 230]+0)/383;c3 = ([120 150 230]+128)/383;patch([0 1 1 0],[0 0 1 1],c1);patch([0 1 1 1-e 1-e 0+e],[0 0 1 1-e 0+e 0+e],c2);patch([0 0 1 1-e 0+e 0+e],[0 1 1 1-e 1-e 0+e],c3);plot([0 1 1 0 0],[0 0 1 1 0]);disp('Weights');
  "IW{1,1}(29,:)'" : Constant  Value=[0.444675412344324560987018912783241830766201019287109375;-1.6313951929328123213736034813337028026580810546875;-0.146802730698376182605358053478994406759738922119140625;-2.349077383159736687190388693124987185001373291015625;1.1679945460990948102875108816078864037990570068359375;1.194565285347806149474081394146196544170379638671875]
      mask Display: e = 0.06;c1 = [120 150 230]/255;c2 = ([120 150 230]+0)/383;c3 = ([120 150 230]+128)/383;patch([0 1 1 0],[0 0 1 1],c1);patch([0 1 1 1-e 1-e 0+e],[0 0 1 1-e 0+e 0+e],c2);patch([0 0 1 1-e 0+e 0+e],[0 1 1 1-e 1-e 0+e],c3);plot([0 1 1 0 0],[0 0 1 1 0]);disp('Weights');
  "IW{1,1}(3,:)'" : Constant  Value=[-0.69051427811071730555880776591948233544826507568359375;-0.216518565497571646716323812142945826053619384765625;-2.062992166029832485918404927360825240612030029296875;-1.8047737650463193670447026306646876037120819091796875;1.638400020802584844403781971777789294719696044921875;-1.0410682488746123564027357133454643189907073974609375]
      mask Display: e = 0.06;c1 = [120 150 230]/255;c2 = ([120 150 230]+0)/383;c3 = ([120 150 230]+128)/383;patch([0 1 1 0],[0 0 1 1],c1);patch([0 1 1 1-e 1-e 0+e],[0 0 1 1-e 0+e 0+e],c2);patch([0 0 1 1-e 0+e 0+e],[0 1 1 1-e 1-e 0+e],c3);plot([0 1 1 0 0],[0 0 1 1 0]);disp('Weights');
  "IW{1,1}(30,:)'" : Constant  Value=[1.5059116051544119141425426278146915137767791748046875;-1.82915564426629639882548872265033423900604248046875;-2.264528317077019181624564225785434246063232421875;-0.584717176190996834606039556092582643032073974609375;-0.58197694404638655729655738468864001333713531494140625;0.152642970894356799771429678003187291324138641357421875]
      mask Display: e = 0.06;c1 = [120 150 230]/255;c2 = ([120 150 230]+0)/383;c3 = ([120 150 230]+128)/383;patch([0 1 1 0],[0 0 1 1],c1);patch([0 1 1 1-e 1-e 0+e],[0 0 1 1-e 0+e 0+e],c2);patch([0 0 1 1-e 0+e 0+e],[0 1 1 1-e 1-e 0+e],c3);plot([0 1 1 0 0],[0 0 1 1 0]);disp('Weights');
  "IW{1,1}(31,:)'" : Constant  Value=[-1.5078543767904488692721542975050397217273712158203125;1.8184771703647830687344821853912435472011566162109375;1.4193697458621332696537820083904080092906951904296875;1.30209326634704414260568228201009333133697509765625;0.21788010677270108761405253972043283283710479736328125;1.253671073360234533566881509614177048206329345703125]
      mask Display: e = 0.06;c1 = [120 150 230]/255;c2 = ([120 150 230]+0)/383;c3 = ([120 150 230]+128)/383;patch([0 1 1 0],[0 0 1 1],c1);patch([0 1 1 1-e 1-e 0+e],[0 0 1 1-e 0+e 0+e],c2);patch([0 0 1 1-e 0+e 0+e],[0 1 1 1-e 1-e 0+e],c3);plot([0 1 1 0 0],[0 0 1 1 0]);disp('Weights');
  "IW{1,1}(32,:)'" : Constant  Value=[0.056303338369500917359733449529812787659466266632080078125;2.326263745671013349891609323094598948955535888671875;-0.360050924841303909840206642911653034389019012451171875;2.36066259608954798210334047325886785984039306640625;-0.63056553780837332201514300322742201387882232666015625;-0.326422516607810131450406743169878609478473663330078125]
      mask Display: e = 0.06;c1 = [120 150 230]/255;c2 = ([120 150 230]+0)/383;c3 = ([120 150 230]+128)/383;patch([0 1 1 0],[0 0 1 1],c1);patch([0 1 1 1-e 1-e 0+e],[0 0 1 1-e 0+e 0+e],c2);patch([0 0 1 1-e 0+e 0+e],[0 1 1 1-e 1-e 0+e],c3);plot([0 1 1 0 0],[0 0 1 1 0]);disp('Weights');
  "IW{1,1}(33,:)'" : Constant  Value=[1.590665928945019569340502130216918885707855224609375;1.986648826272325418784703288110904395580291748046875;1.04432787633591406262212331057526171207427978515625;-1.639946020887993238801527695613913238048553466796875;0.88046324798329578253941463117371313273906707763671875;-0.7562893118162647976276957706431858241558074951171875]
      mask Display: e = 0.06;c1 = [120 150 230]/255;c2 = ([120 150 230]+0)/383;c3 = ([120 150 230]+128)/383;patch([0 1 1 0],[0 0 1 1],c1);patch([0 1 1 1-e 1-e 0+e],[0 0 1 1-e 0+e 0+e],c2);patch([0 0 1 1-e 0+e 0+e],[0 1 1 1-e 1-e 0+e],c3);plot([0 1 1 0 0],[0 0 1 1 0]);disp('Weights');
  "IW{1,1}(34,:)'" : Constant  Value=[-0.7594529398829326094499947430449537932872772216796875;1.6309414075747714623076944917556829750537872314453125;-0.9304192129677806288867714101797901093959808349609375;1.2895877391092920305482039111666381359100341796875;1.1296101255452144496160826747654937207698822021484375;-1.9702095189396866548037223765277303755283355712890625]
      mask Display: e = 0.06;c1 = [120 150 230]/255;c2 = ([120 150 230]+0)/383;c3 = ([120 150 230]+128)/383;patch([0 1 1 0],[0 0 1 1],c1);patch([0 1 1 1-e 1-e 0+e],[0 0 1 1-e 0+e 0+e],c2);patch([0 0 1 1-e 0+e 0+e],[0 1 1 1-e 1-e 0+e],c3);plot([0 1 1 0 0],[0 0 1 1 0]);disp('Weights');
  "IW{1,1}(35,:)'" : Constant  Value=[-1.5083470337215179046808088969555683434009552001953125;-1.3190456214974430881881062305183149874210357666015625;0.975747947120767289419518419890664517879486083984375;1.8802805800480495435067496146075427532196044921875;-0.4059182125293199216997663825168274343013763427734375;1.707088410201985428926718668662942945957183837890625]
      mask Display: e = 0.06;c1 = [120 150 230]/255;c2 = ([120 150 230]+0)/383;c3 = ([120 150 230]+128)/383;patch([0 1 1 0],[0 0 1 1],c1);patch([0 1 1 1-e 1-e 0+e],[0 0 1 1-e 0+e 0+e],c2);patch([0 0 1 1-e 0+e 0+e],[0 1 1 1-e 1-e 0+e],c3);plot([0 1 1 0 0],[0 0 1 1 0]);disp('Weights');
  "IW{1,1}(36,:)'" : Constant  Value=[0.9070173529557543634638250296120531857013702392578125;1.639723669164388386576547418371774256229400634765625;0.4258596423072338321702545727021060883998870849609375;1.9266158391495762369771682642749510705471038818359375;-0.4724909821622997885270933693391270935535430908203125;-1.987438206343103974660380117711611092090606689453125]
      mask Display: e = 0.06;c1 = [120 150 230]/255;c2 = ([120 150 230]+0)/383;c3 = ([120 150 230]+128)/383;patch([0 1 1 0],[0 0 1 1],c1);patch([0 1 1 1-e 1-e 0+e],[0 0 1 1-e 0+e 0+e],c2);patch([0 0 1 1-e 0+e 0+e],[0 1 1 1-e 1-e 0+e],c3);plot([0 1 1 0 0],[0 0 1 1 0]);disp('Weights');
  "IW{1,1}(37,:)'" : Constant  Value=[-2.05193222093290383867270065820775926113128662109375;-0.239783119171963932103608385659754276275634765625;0.364549175391427227044260916954954154789447784423828125;-2.464970385382296402809743085526861250400543212890625;-0.79282557028343270122405783695285208523273468017578125;-0.96184761508954486064482125584618188440799713134765625]
      mask Display: e = 0.06;c1 = [120 150 230]/255;c2 = ([120 150 230]+0)/383;c3 = ([120 150 230]+128)/383;patch([0 1 1 0],[0 0 1 1],c1);patch([0 1 1 1-e 1-e 0+e],[0 0 1 1-e 0+e 0+e],c2);patch([0 0 1 1-e 0+e 0+e],[0 1 1 1-e 1-e 0+e],c3);plot([0 1 1 0 0],[0 0 1 1 0]);disp('Weights');
  "IW{1,1}(38,:)'" : Constant  Value=[1.1597461912509630099776813949574716389179229736328125;1.4769994564052648655660959775559604167938232421875;0.5320256707110768701340930419974029064178466796875;-1.9179502438771482974999571524676866829395294189453125;1.2205751905258306333479367822292260825634002685546875;-1.5790784779995046260836488727363757789134979248046875]
      mask Display: e = 0.06;c1 = [120 150 230]/255;c2 = ([120 150 230]+0)/383;c3 = ([120 150 230]+128)/383;patch([0 1 1 0],[0 0 1 1],c1);patch([0 1 1 1-e 1-e 0+e],[0 0 1 1-e 0+e 0+e],c2);patch([0 0 1 1-e 0+e 0+e],[0 1 1 1-e 1-e 0+e],c3);plot([0 1 1 0 0],[0 0 1 1 0]);disp('Weights');
  "IW{1,1}(39,:)'" : Constant  Value=[0.98990204803341885764211838250048458576202392578125;-2.02893680276332855072496386128477752208709716796875;-1.695822120139938160576775771914981305599212646484375;-0.1087232837825185816083006784538156352937221527099609375;-1.8307849433666081306881778800743632018566131591796875;0.43725035302258696834343254522536881268024444580078125]
      mask Display: e = 0.06;c1 = [120 150 230]/255;c2 = ([120 150 230]+0)/383;c3 = ([120 150 230]+128)/383;patch([0 1 1 0],[0 0 1 1],c1);patch([0 1 1 1-e 1-e 0+e],[0 0 1 1-e 0+e 0+e],c2);patch([0 0 1 1-e 0+e 0+e],[0 1 1 1-e 1-e 0+e],c3);plot([0 1 1 0 0],[0 0 1 1 0]);disp('Weights');
  "IW{1,1}(4,:)'" : Constant  Value=[-1.400665535021616836530711225350387394428253173828125;-1.001004546158948738110439080628566443920135498046875;0.65839017391376863930219087706063874065876007080078125;-1.3568414241650386120596749606193043291568756103515625;-1.6408803473394950600550146191380918025970458984375;1.7641771317316135014863220931147225201129913330078125]
      mask Display: e = 0.06;c1 = [120 150 230]/255;c2 = ([120 150 230]+0)/383;c3 = ([120 150 230]+128)/383;patch([0 1 1 0],[0 0 1 1],c1);patch([0 1 1 1-e 1-e 0+e],[0 0 1 1-e 0+e 0+e],c2);patch([0 0 1 1-e 0+e 0+e],[0 1 1 1-e 1-e 0+e],c3);plot([0 1 1 0 0],[0 0 1 1 0]);disp('Weights');
  "IW{1,1}(40,:)'" : Constant  Value=[1.9027288981742522810947093603317625820636749267578125;-1.061096351806102067172332681366242468357086181640625;0.94426071865080440925765969950589351356029510498046875;0.79671270190230225605176883618696592748165130615234375;0.67145185705094390105074353414238430559635162353515625;2.1204202193168324441785443923436105251312255859375]
      mask Display: e = 0.06;c1 = [120 150 230]/255;c2 = ([120 150 230]+0)/383;c3 = ([120 150 230]+128)/383;patch([0 1 1 0],[0 0 1 1],c1);patch([0 1 1 1-e 1-e 0+e],[0 0 1 1-e 0+e 0+e],c2);patch([0 0 1 1-e 0+e 0+e],[0 1 1 1-e 1-e 0+e],c3);plot([0 1 1 0 0],[0 0 1 1 0]);disp('Weights');
  "IW{1,1}(41,:)'" : Constant  Value=[1.743188562898662752331802039407193660736083984375;-0.81033777604370393898847169111832045018672943115234375;-0.078347869727921348736998652384500019252300262451171875;-1.904579973101975465255009112297557294368743896484375;1.978992071959944976100587155087850987911224365234375;-0.44888980476028683685996156782493926584720611572265625]
      mask Display: e = 0.06;c1 = [120 150 230]/255;c2 = ([120 150 230]+0)/383;c3 = ([120 150 230]+128)/383;patch([0 1 1 0],[0 0 1 1],c1);patch([0 1 1 1-e 1-e 0+e],[0 0 1 1-e 0+e 0+e],c2);patch([0 0 1 1-e 0+e 0+e],[0 1 1 1-e 1-e 0+e],c3);plot([0 1 1 0 0],[0 0 1 1 0]);disp('Weights');
  "IW{1,1}(42,:)'" : Constant  Value=[-0.68406238691575094179597726906649768352508544921875;-0.99200724518382676908601069953874684870243072509765625;0.96868153371503196158442960950196720659732818603515625;-1.9651037971238471957491356079117394983768463134765625;1.2066707516121948362552984690410085022449493408203125;1.9356187927450225760850344158825464546680450439453125]
      mask Display: e = 0.06;c1 = [120 150 230]/255;c2 = ([120 150 230]+0)/383;c3 = ([120 150 230]+128)/383;patch([0 1 1 0],[0 0 1 1],c1);patch([0 1 1 1-e 1-e 0+e],[0 0 1 1-e 0+e 0+e],c2);patch([0 0 1 1-e 0+e 0+e],[0 1 1 1-e 1-e 0+e],c3);plot([0 1 1 0 0],[0 0 1 1 0]);disp('Weights');
  "IW{1,1}(43,:)'" : Constant  Value=[-1.925743079831698789661231785430572926998138427734375;1.4325343043730500713905939846881665289402008056640625;-0.56103182753329272625109069849713705480098724365234375;-1.8645073589926359769464170312858186662197113037109375;-1.4675880949608661740768411618773825466632843017578125;-0.337538646804358688502389895802480168640613555908203125]
      mask Display: e = 0.06;c1 = [120 150 230]/255;c2 = ([120 150 230]+0)/383;c3 = ([120 150 230]+128)/383;patch([0 1 1 0],[0 0 1 1],c1);patch([0 1 1 1-e 1-e 0+e],[0 0 1 1-e 0+e 0+e],c2);patch([0 0 1 1-e 0+e 0+e],[0 1 1 1-e 1-e 0+e],c3);plot([0 1 1 0 0],[0 0 1 1 0]);disp('Weights');
  "IW{1,1}(44,:)'" : Constant  Value=[0.92353013177371490183276137031498365104198455810546875;0.1640574696507697549652249335849774070084095001220703125;-0.1536944791850582969772176511469297111034393310546875;2.069457057570132985091504451702348887920379638671875;0.2356358858732525984880368241647374816238880157470703125;2.400771357558455054714841025997884571552276611328125]
      mask Display: e = 0.06;c1 = [120 150 230]/255;c2 = ([120 150 230]+0)/383;c3 = ([120 150 230]+128)/383;patch([0 1 1 0],[0 0 1 1],c1);patch([0 1 1 1-e 1-e 0+e],[0 0 1 1-e 0+e 0+e],c2);patch([0 0 1 1-e 0+e 0+e],[0 1 1 1-e 1-e 0+e],c3);plot([0 1 1 0 0],[0 0 1 1 0]);disp('Weights');
  "IW{1,1}(45,:)'" : Constant  Value=[-2.17652553879322940844076583744026720523834228515625;-1.1768906623808035316613995746592991054058074951171875;1.1482566059150622894691196052008308470249176025390625;-1.72672547597881465009095336426980793476104736328125;0.485446845502492896340385186704224906861782073974609375;-0.3821136726546023876238677985384128987789154052734375]
      mask Display: e = 0.06;c1 = [120 150 230]/255;c2 = ([120 150 230]+0)/383;c3 = ([120 150 230]+128)/383;patch([0 1 1 0],[0 0 1 1],c1);patch([0 1 1 1-e 1-e 0+e],[0 0 1 1-e 0+e 0+e],c2);patch([0 0 1 1-e 0+e 0+e],[0 1 1 1-e 1-e 0+e],c3);plot([0 1 1 0 0],[0 0 1 1 0]);disp('Weights');
  "IW{1,1}(46,:)'" : Constant  Value=[-0.05586132479323814570282280556057230569422245025634765625;-0.1485475828829773414785364593626582063734531402587890625;2.374173493729571315924431473831646144390106201171875;-0.72611326493300565321220574332983233034610748291015625;0.02572592585623301175701271858997642993927001953125;-2.225659697063075981304791639558970928192138671875]
      mask Display: e = 0.06;c1 = [120 150 230]/255;c2 = ([120 150 230]+0)/383;c3 = ([120 150 230]+128)/383;patch([0 1 1 0],[0 0 1 1],c1);patch([0 1 1 1-e 1-e 0+e],[0 0 1 1-e 0+e 0+e],c2);patch([0 0 1 1-e 0+e 0+e],[0 1 1 1-e 1-e 0+e],c3);plot([0 1 1 0 0],[0 0 1 1 0]);disp('Weights');
  "IW{1,1}(47,:)'" : Constant  Value=[-0.428403932812163545928996200018445961177349090576171875;1.31000332897173077384422867908142507076263427734375;2.49075399944490083470327590475790202617645263671875;-0.7078833296508924011192220859811641275882720947265625;-0.9178813698696191014647638439782895147800445556640625;1.4525878875317961291813162461039610207080841064453125]
      mask Display: e = 0.06;c1 = [120 150 230]/255;c2 = ([120 150 230]+0)/383;c3 = ([120 150 230]+128)/383;patch([0 1 1 0],[0 0 1 1],c1);patch([0 1 1 1-e 1-e 0+e],[0 0 1 1-e 0+e 0+e],c2);patch([0 0 1 1-e 0+e 0+e],[0 1 1 1-e 1-e 0+e],c3);plot([0 1 1 0 0],[0 0 1 1 0]);disp('Weights');
  "IW{1,1}(48,:)'" : Constant  Value=[-0.9742839338042721397670220540021546185016632080078125;-0.52148405634120920115748276657541282474994659423828125;2.324441230921293399802607382298447191715240478515625;0.56308867095570536154269802864291705191135406494140625;-2.066962809368611875271426470135338604450225830078125;-1.35596593097343198763837790465913712978363037109375]
      mask Display: e = 0.06;c1 = [120 150 230]/255;c2 = ([120 150 230]+0)/383;c3 = ([120 150 230]+128)/383;patch([0 1 1 0],[0 0 1 1],c1);patch([0 1 1 1-e 1-e 0+e],[0 0 1 1-e 0+e 0+e],c2);patch([0 0 1 1-e 0+e 0+e],[0 1 1 1-e 1-e 0+e],c3);plot([0 1 1 0 0],[0 0 1 1 0]);disp('Weights');
  "IW{1,1}(49,:)'" : Constant  Value=[0.79596428631687710097963872613036073744297027587890625;0.90705481475542304448111963210976682603359222412109375;2.596297912995901402410936498199589550495147705078125;-0.392030868206213300997120541069307364523410797119140625;-1.3537654010271291671330118333571590483188629150390625;1.1925025927884471688145140433334745466709136962890625]
      mask Display: e = 0.06;c1 = [120 150 230]/255;c2 = ([120 150 230]+0)/383;c3 = ([120 150 230]+128)/383;patch([0 1 1 0],[0 0 1 1],c1);patch([0 1 1 1-e 1-e 0+e],[0 0 1 1-e 0+e 0+e],c2);patch([0 0 1 1-e 0+e 0+e],[0 1 1 1-e 1-e 0+e],c3);plot([0 1 1 0 0],[0 0 1 1 0]);disp('Weights');
  "IW{1,1}(5,:)'" : Constant  Value=[-1.6812091311831574014235002323403023183345794677734375;-2.099013561536460681367088909610174596309661865234375;-0.138449048774836658282083590165711939334869384765625;-0.255043831988231273211198413264355622231960296630859375;-0.82697557283357225887954200516105629503726959228515625;1.805693036629701708761785994283854961395263671875]
      mask Display: e = 0.06;c1 = [120 150 230]/255;c2 = ([120 150 230]+0)/383;c3 = ([120 150 230]+128)/383;patch([0 1 1 0],[0 0 1 1],c1);patch([0 1 1 1-e 1-e 0+e],[0 0 1 1-e 0+e 0+e],c2);patch([0 0 1 1-e 0+e 0+e],[0 1 1 1-e 1-e 0+e],c3);plot([0 1 1 0 0],[0 0 1 1 0]);disp('Weights');
  "IW{1,1}(50,:)'" : Constant  Value=[0.89486633044997965225064717742498032748699188232421875;-1.1192906420108219567310925413039512932300567626953125;1.413550257349271532802958972752094268798828125;1.17429501671708091947721186443231999874114990234375;2.11930605520489390158900278038345277309417724609375;1.2929933465378018464519982444471679627895355224609375]
      mask Display: e = 0.06;c1 = [120 150 230]/255;c2 = ([120 150 230]+0)/383;c3 = ([120 150 230]+128)/383;patch([0 1 1 0],[0 0 1 1],c1);patch([0 1 1 1-e 1-e 0+e],[0 0 1 1-e 0+e 0+e],c2);patch([0 0 1 1-e 0+e 0+e],[0 1 1 1-e 1-e 0+e],c3);plot([0 1 1 0 0],[0 0 1 1 0]);disp('Weights');
  "IW{1,1}(51,:)'" : Constant  Value=[-0.043308723363899563618684140919867786578834056854248046875;-2.316464429770070498904033229337073862552642822265625;-1.142808383933779037278100076946429908275604248046875;-1.2962743008336283789816434364183805882930755615234375;0.2731835615020177243650323362089693546295166015625;-1.69710160267660281618873341358266770839691162109375]
      mask Display: e = 0.06;c1 = [120 150 230]/255;c2 = ([120 150 230]+0)/383;c3 = ([120 150 230]+128)/383;patch([0 1 1 0],[0 0 1 1],c1);patch([0 1 1 1-e 1-e 0+e],[0 0 1 1-e 0+e 0+e],c2);patch([0 0 1 1-e 0+e 0+e],[0 1 1 1-e 1-e 0+e],c3);plot([0 1 1 0 0],[0 0 1 1 0]);disp('Weights');
  "IW{1,1}(52,:)'" : Constant  Value=[-1.6705217985822871096246444722055457532405853271484375;1.672549650490540162905972465523518621921539306640625;1.646687519863998971914043067954480648040771484375;-0.456164231515113705039965452670003287494182586669921875;-0.686728347251520876426411632564850151538848876953125;-1.5450051069341756981856406127917580306529998779296875]
      mask Display: e = 0.06;c1 = [120 150 230]/255;c2 = ([120 150 230]+0)/383;c3 = ([120 150 230]+128)/383;patch([0 1 1 0],[0 0 1 1],c1);patch([0 1 1 1-e 1-e 0+e],[0 0 1 1-e 0+e 0+e],c2);patch([0 0 1 1-e 0+e 0+e],[0 1 1 1-e 1-e 0+e],c3);plot([0 1 1 0 0],[0 0 1 1 0]);disp('Weights');
  "IW{1,1}(53,:)'" : Constant  Value=[1.7691688804561598313824788419879041612148284912109375;1.3597081898468366123466921635554172098636627197265625;1.886369234568373798310858546756207942962646484375;-0.4383101819727670545034925453364849090576171875;1.477533073799634610878683815826661884784698486328125;0.7143948186490816087967914427281357347965240478515625]
      mask Display: e = 0.06;c1 = [120 150 230]/255;c2 = ([120 150 230]+0)/383;c3 = ([120 150 230]+128)/383;patch([0 1 1 0],[0 0 1 1],c1);patch([0 1 1 1-e 1-e 0+e],[0 0 1 1-e 0+e 0+e],c2);patch([0 0 1 1-e 0+e 0+e],[0 1 1 1-e 1-e 0+e],c3);plot([0 1 1 0 0],[0 0 1 1 0]);disp('Weights');
  "IW{1,1}(54,:)'" : Constant  Value=[-1.5657549445941281174299319900455884635448455810546875;2.61012386851933797515812329947948455810546875;1.1570084044857196214906025488744489848613739013671875;0.0749735851759605054223101205934653989970684051513671875;-0.76279691722436793188677484067738987505435943603515625;-0.49571437410235807963232446127221919596195220947265625]
      mask Display: e = 0.06;c1 = [120 150 230]/255;c2 = ([120 150 230]+0)/383;c3 = ([120 150 230]+128)/383;patch([0 1 1 0],[0 0 1 1],c1);patch([0 1 1 1-e 1-e 0+e],[0 0 1 1-e 0+e 0+e],c2);patch([0 0 1 1-e 0+e 0+e],[0 1 1 1-e 1-e 0+e],c3);plot([0 1 1 0 0],[0 0 1 1 0]);disp('Weights');
  "IW{1,1}(55,:)'" : Constant  Value=[0.9674623114421370129178967545158229768276214599609375;2.008586885882824635274346292135305702686309814453125;-0.44703713736385441990250910748727619647979736328125;1.5991377202775234334097831379040144383907318115234375;-1.447760269687393464010938259889371693134307861328125;-1.1270961725126509289651721701375208795070648193359375]
      mask Display: e = 0.06;c1 = [120 150 230]/255;c2 = ([120 150 230]+0)/383;c3 = ([120 150 230]+128)/383;patch([0 1 1 0],[0 0 1 1],c1);patch([0 1 1 1-e 1-e 0+e],[0 0 1 1-e 0+e 0+e],c2);patch([0 0 1 1-e 0+e 0+e],[0 1 1 1-e 1-e 0+e],c3);plot([0 1 1 0 0],[0 0 1 1 0]);disp('Weights');
  "IW{1,1}(56,:)'" : Constant  Value=[-1.74641650679039361904187899199314415454864501953125;0.053932515036601014202233272953890264034271240234375;-1.6117449720831069637227983548655174672603607177734375;-1.70038386629396764959665233618579804897308349609375;-1.68702265382542559990497466060332953929901123046875;-0.380665522184446436515514733400777913630008697509765625]
      mask Display: e = 0.06;c1 = [120 150 230]/255;c2 = ([120 150 230]+0)/383;c3 = ([120 150 230]+128)/383;patch([0 1 1 0],[0 0 1 1],c1);patch([0 1 1 1-e 1-e 0+e],[0 0 1 1-e 0+e 0+e],c2);patch([0 0 1 1-e 0+e 0+e],[0 1 1 1-e 1-e 0+e],c3);plot([0 1 1 0 0],[0 0 1 1 0]);disp('Weights');
  "IW{1,1}(57,:)'" : Constant  Value=[-0.81905007531019202726696448735310696065425872802734375;0.6996483589727076068953692811192013323307037353515625;-1.8890610072295845878187492417055182158946990966796875;-1.4976395144216325672203993235598318278789520263671875;-1.8762714147460382019261260211351327598094940185546875;-0.93291564540283544726406717018107883632183074951171875]
      mask Display: e = 0.06;c1 = [120 150 230]/255;c2 = ([120 150 230]+0)/383;c3 = ([120 150 230]+128)/383;patch([0 1 1 0],[0 0 1 1],c1);patch([0 1 1 1-e 1-e 0+e],[0 0 1 1-e 0+e 0+e],c2);patch([0 0 1 1-e 0+e 0+e],[0 1 1 1-e 1-e 0+e],c3);plot([0 1 1 0 0],[0 0 1 1 0]);disp('Weights');
  "IW{1,1}(58,:)'" : Constant  Value=[-1.8805624425166451718638427337282337248325347900390625;-1.495554185007188063849525860860012471675872802734375;1.8234602821998275867798611216130666434764862060546875;1.00091416719776216126547296880744397640228271484375;-0.9512975687287965609328921345877461135387420654296875;-0.64823750609684349655026380787603557109832763671875]
      mask Display: e = 0.06;c1 = [120 150 230]/255;c2 = ([120 150 230]+0)/383;c3 = ([120 150 230]+128)/383;patch([0 1 1 0],[0 0 1 1],c1);patch([0 1 1 1-e 1-e 0+e],[0 0 1 1-e 0+e 0+e],c2);patch([0 0 1 1-e 0+e 0+e],[0 1 1 1-e 1-e 0+e],c3);plot([0 1 1 0 0],[0 0 1 1 0]);disp('Weights');
  "IW{1,1}(59,:)'" : Constant  Value=[-1.6669685514965102424156384586240164935588836669921875;0.9498958910809089939419891379657201468944549560546875;1.8515859521765005712978791052591986954212188720703125;1.5474591613284010005457957959151826798915863037109375;1.3949691649206348298406510366476140916347503662109375;0.0745251371340933388420779692751239053905010223388671875]
      mask Display: e = 0.06;c1 = [120 150 230]/255;c2 = ([120 150 230]+0)/383;c3 = ([120 150 230]+128)/383;patch([0 1 1 0],[0 0 1 1],c1);patch([0 1 1 1-e 1-e 0+e],[0 0 1 1-e 0+e 0+e],c2);patch([0 0 1 1-e 0+e 0+e],[0 1 1 1-e 1-e 0+e],c3);plot([0 1 1 0 0],[0 0 1 1 0]);disp('Weights');
  "IW{1,1}(6,:)'" : Constant  Value=[-2.1917197621474997504265047609806060791015625;0.7485016830457655867547828165697865188121795654296875;-0.2300630687697424736626317098853178322315216064453125;-1.8029103977364389077564510444062761962413787841796875;-1.6223573045062116282366559971706010401248931884765625;1.200408884481185989301366134895943105220794677734375]
      mask Display: e = 0.06;c1 = [120 150 230]/255;c2 = ([120 150 230]+0)/383;c3 = ([120 150 230]+128)/383;patch([0 1 1 0],[0 0 1 1],c1);patch([0 1 1 1-e 1-e 0+e],[0 0 1 1-e 0+e 0+e],c2);patch([0 0 1 1-e 0+e 0+e],[0 1 1 1-e 1-e 0+e],c3);plot([0 1 1 0 0],[0 0 1 1 0]);disp('Weights');
  "IW{1,1}(60,:)'" : Constant  Value=[-1.2958964496119815823504950458300299942493438720703125;1.4015116728669330115053526242263615131378173828125;1.6559620982796630084266098492662422358989715576171875;1.759951808462708822133890862460248172283172607421875;0.82803181224727884224279250702238641679286956787109375;-1.142290134116260791330432766699232161045074462890625]
      mask Display: e = 0.06;c1 = [120 150 230]/255;c2 = ([120 150 230]+0)/383;c3 = ([120 150 230]+128)/383;patch([0 1 1 0],[0 0 1 1],c1);patch([0 1 1 1-e 1-e 0+e],[0 0 1 1-e 0+e 0+e],c2);patch([0 0 1 1-e 0+e 0+e],[0 1 1 1-e 1-e 0+e],c3);plot([0 1 1 0 0],[0 0 1 1 0]);disp('Weights');
  "IW{1,1}(61,:)'" : Constant  Value=[1.365457975519275723996770466328598558902740478515625;-0.08679708376644930389876009257932309992611408233642578125;-1.602686800156860602584174557705409824848175048828125;1.6017670835552724195594009870546869933605194091796875;1.2795847190128635251227251501404680311679840087890625;1.554233115761079364602892383118160068988800048828125]
      mask Display: e = 0.06;c1 = [120 150 230]/255;c2 = ([120 150 230]+0)/383;c3 = ([120 150 230]+128)/383;patch([0 1 1 0],[0 0 1 1],c1);patch([0 1 1 1-e 1-e 0+e],[0 0 1 1-e 0+e 0+e],c2);patch([0 0 1 1-e 0+e 0+e],[0 1 1 1-e 1-e 0+e],c3);plot([0 1 1 0 0],[0 0 1 1 0]);disp('Weights');
  "IW{1,1}(62,:)'" : Constant  Value=[0.65507917565954809635542233081650920212268829345703125;1.86927921783895190088742310763336718082427978515625;-0.09609002785223559606198051596948062069714069366455078125;1.118453075536961716096584495971910655498504638671875;1.87530712438396829355724548804573714733123779296875;-1.67335815593133485634780299733392894268035888671875]
      mask Display: e = 0.06;c1 = [120 150 230]/255;c2 = ([120 150 230]+0)/383;c3 = ([120 150 230]+128)/383;patch([0 1 1 0],[0 0 1 1],c1);patch([0 1 1 1-e 1-e 0+e],[0 0 1 1-e 0+e 0+e],c2);patch([0 0 1 1-e 0+e 0+e],[0 1 1 1-e 1-e 0+e],c3);plot([0 1 1 0 0],[0 0 1 1 0]);disp('Weights');
  "IW{1,1}(63,:)'" : Constant  Value=[-0.82798579406719918782897593700909055769443511962890625;-1.94446761499597986500020851963199675083160400390625;0.285147522219315219249580195537419058382511138916015625;2.508521516549361063397327598067931830883026123046875;-0.35551416935848012546017571366974152624607086181640625;-0.90702661434517040106584317982196807861328125]
      mask Display: e = 0.06;c1 = [120 150 230]/255;c2 = ([120 150 230]+0)/383;c3 = ([120 150 230]+128)/383;patch([0 1 1 0],[0 0 1 1],c1);patch([0 1 1 1-e 1-e 0+e],[0 0 1 1-e 0+e 0+e],c2);patch([0 0 1 1-e 0+e 0+e],[0 1 1 1-e 1-e 0+e],c3);plot([0 1 1 0 0],[0 0 1 1 0]);disp('Weights');
  "IW{1,1}(64,:)'" : Constant  Value=[2.288883723726093055717001334414817392826080322265625;1.2463141055459765471624677957152016460895538330078125;0.999261368088907975248957882286049425601959228515625;-1.6160044314867203496532965800724923610687255859375;-0.004221568845972877015437774161910056136548519134521484375;-1.0137252544997912284685526174143888056278228759765625]
      mask Display: e = 0.06;c1 = [120 150 230]/255;c2 = ([120 150 230]+0)/383;c3 = ([120 150 230]+128)/383;patch([0 1 1 0],[0 0 1 1],c1);patch([0 1 1 1-e 1-e 0+e],[0 0 1 1-e 0+e 0+e],c2);patch([0 0 1 1-e 0+e 0+e],[0 1 1 1-e 1-e 0+e],c3);plot([0 1 1 0 0],[0 0 1 1 0]);disp('Weights');
  "IW{1,1}(65,:)'" : Constant  Value=[-1.656444112360414777640471584163606166839599609375;-1.150465858655772333207778501673601567745208740234375;-0.57299525264213702069326927812653593719005584716796875;1.882177298587697666931717321858741343021392822265625;-1.822176593409476907936550560407340526580810546875;-0.2011660988971795405166886894221534021198749542236328125]
      mask Display: e = 0.06;c1 = [120 150 230]/255;c2 = ([120 150 230]+0)/383;c3 = ([120 150 230]+128)/383;patch([0 1 1 0],[0 0 1 1],c1);patch([0 1 1 1-e 1-e 0+e],[0 0 1 1-e 0+e 0+e],c2);patch([0 0 1 1-e 0+e 0+e],[0 1 1 1-e 1-e 0+e],c3);plot([0 1 1 0 0],[0 0 1 1 0]);disp('Weights');
  "IW{1,1}(66,:)'" : Constant  Value=[0.07978661994161172221762257095178938470780849456787109375;1.212335296025150110921231316751800477504730224609375;0.949508328538817725217313636676408350467681884765625;-0.72068583112134121382297280433704145252704620361328125;2.649265770566450850509454539860598742961883544921875;-1.4095368307951681163814328101580031216144561767578125]
      mask Display: e = 0.06;c1 = [120 150 230]/255;c2 = ([120 150 230]+0)/383;c3 = ([120 150 230]+128)/383;patch([0 1 1 0],[0 0 1 1],c1);patch([0 1 1 1-e 1-e 0+e],[0 0 1 1-e 0+e 0+e],c2);patch([0 0 1 1-e 0+e 0+e],[0 1 1 1-e 1-e 0+e],c3);plot([0 1 1 0 0],[0 0 1 1 0]);disp('Weights');
  "IW{1,1}(67,:)'" : Constant  Value=[1.38147356552817601738070152350701391696929931640625;2.026036236984963156970707132131792604923248291015625;-0.307902552955303387971497386388364247977733612060546875;-1.6236951982282088469133896069251932203769683837890625;-0.74640253180175519798211780653218738734722137451171875;1.5272051119882299463625940916244871914386749267578125]
      mask Display: e = 0.06;c1 = [120 150 230]/255;c2 = ([120 150 230]+0)/383;c3 = ([120 150 230]+128)/383;patch([0 1 1 0],[0 0 1 1],c1);patch([0 1 1 1-e 1-e 0+e],[0 0 1 1-e 0+e 0+e],c2);patch([0 0 1 1-e 0+e 0+e],[0 1 1 1-e 1-e 0+e],c3);plot([0 1 1 0 0],[0 0 1 1 0]);disp('Weights');
  "IW{1,1}(68,:)'" : Constant  Value=[1.2699501341865662151775495658512227237224578857421875;-2.35095266848429584882751441909931600093841552734375;0.7562403843777525391800509169115684926509857177734375;-1.9420788456999691362625526380725204944610595703125;-0.0131240072532986563891288511740640387870371341705322265625;0.0361723624501842089262737545141135342419147491455078125]
      mask Display: e = 0.06;c1 = [120 150 230]/255;c2 = ([120 150 230]+0)/383;c3 = ([120 150 230]+128)/383;patch([0 1 1 0],[0 0 1 1],c1);patch([0 1 1 1-e 1-e 0+e],[0 0 1 1-e 0+e 0+e],c2);patch([0 0 1 1-e 0+e 0+e],[0 1 1 1-e 1-e 0+e],c3);plot([0 1 1 0 0],[0 0 1 1 0]);disp('Weights');
  "IW{1,1}(69,:)'" : Constant  Value=[0.6340530450152248587158965165144763886928558349609375;2.589429502420146800290012834011577069759368896484375;-1.6812788551726882690928732699831016361713409423828125;0.336619632789916523041284790451754815876483917236328125;0.6185855515926246273039623702061362564563751220703125;-0.9902552836211018227885460873949341475963592529296875]
      mask Display: e = 0.06;c1 = [120 150 230]/255;c2 = ([120 150 230]+0)/383;c3 = ([120 150 230]+128)/383;patch([0 1 1 0],[0 0 1 1],c1);patch([0 1 1 1-e 1-e 0+e],[0 0 1 1-e 0+e 0+e],c2);patch([0 0 1 1-e 0+e 0+e],[0 1 1 1-e 1-e 0+e],c3);plot([0 1 1 0 0],[0 0 1 1 0]);disp('Weights');
  "IW{1,1}(7,:)'" : Constant  Value=[1.0898522772478174136523421111633069813251495361328125;2.115389468062768063560952214174903929233551025390625;-0.44381390934335362974394456614390946924686431884765625;-0.37877688994535529953822106108418665826320648193359375;-2.325263246184055443421812015003524720668792724609375;0.69835319788909100413576425125938840210437774658203125]
      mask Display: e = 0.06;c1 = [120 150 230]/255;c2 = ([120 150 230]+0)/383;c3 = ([120 150 230]+128)/383;patch([0 1 1 0],[0 0 1 1],c1);patch([0 1 1 1-e 1-e 0+e],[0 0 1 1-e 0+e 0+e],c2);patch([0 0 1 1-e 0+e 0+e],[0 1 1 1-e 1-e 0+e],c3);plot([0 1 1 0 0],[0 0 1 1 0]);disp('Weights');
  "IW{1,1}(70,:)'" : Constant  Value=[-1.6179090989305227044070534248021431267261505126953125;-1.65198373731971148714592345640994608402252197265625;1.1585825893493859606309115406475029885768890380859375;-1.324092634979123328520245195250026881694793701171875;0.428310434618602464684755659618531353771686553955078125;1.71454750004198075430394965223968029022216796875]
      mask Display: e = 0.06;c1 = [120 150 230]/255;c2 = ([120 150 230]+0)/383;c3 = ([120 150 230]+128)/383;patch([0 1 1 0],[0 0 1 1],c1);patch([0 1 1 1-e 1-e 0+e],[0 0 1 1-e 0+e 0+e],c2);patch([0 0 1 1-e 0+e 0+e],[0 1 1 1-e 1-e 0+e],c3);plot([0 1 1 0 0],[0 0 1 1 0]);disp('Weights');
  "IW{1,1}(71,:)'" : Constant  Value=[0.56415578070913541264275181674747727811336517333984375;0.055531947896769025263541408321543713100254535675048828125;-0.209928495739712117629238719018758274614810943603515625;-2.20347121447011407013860662118531763553619384765625;-2.509768809082769447371674687019549310207366943359375;-0.326825891067102969334001727474969811737537384033203125]
      mask Display: e = 0.06;c1 = [120 150 230]/255;c2 = ([120 150 230]+0)/383;c3 = ([120 150 230]+128)/383;patch([0 1 1 0],[0 0 1 1],c1);patch([0 1 1 1-e 1-e 0+e],[0 0 1 1-e 0+e 0+e],c2);patch([0 0 1 1-e 0+e 0+e],[0 1 1 1-e 1-e 0+e],c3);plot([0 1 1 0 0],[0 0 1 1 0]);disp('Weights');
  "IW{1,1}(72,:)'" : Constant  Value=[1.6137223001440694769570427524740807712078094482421875;-0.68600517057965848533029884492862038314342498779296875;-0.68227255489896965201523926225490868091583251953125;0.76124571475842139900436222887947224080562591552734375;1.2374787759602601244779407352325506508350372314453125;2.4856405133679597696527707739733159542083740234375]
      mask Display: e = 0.06;c1 = [120 150 230]/255;c2 = ([120 150 230]+0)/383;c3 = ([120 150 230]+128)/383;patch([0 1 1 0],[0 0 1 1],c1);patch([0 1 1 1-e 1-e 0+e],[0 0 1 1-e 0+e 0+e],c2);patch([0 0 1 1-e 0+e 0+e],[0 1 1 1-e 1-e 0+e],c3);plot([0 1 1 0 0],[0 0 1 1 0]);disp('Weights');
  "IW{1,1}(73,:)'" : Constant  Value=[-1.03150207891426504147602827288210391998291015625;-1.288082405712043243539710601908154785633087158203125;-1.4777253276427912975776735038380138576030731201171875;1.901927174663900377282743647811003029346466064453125;1.3753834529990600632487485199817456305027008056640625;0.96308916793399645950302101482520811259746551513671875]
      mask Display: e = 0.06;c1 = [120 150 230]/255;c2 = ([120 150 230]+0)/383;c3 = ([120 150 230]+128)/383;patch([0 1 1 0],[0 0 1 1],c1);patch([0 1 1 1-e 1-e 0+e],[0 0 1 1-e 0+e 0+e],c2);patch([0 0 1 1-e 0+e 0+e],[0 1 1 1-e 1-e 0+e],c3);plot([0 1 1 0 0],[0 0 1 1 0]);disp('Weights');
  "IW{1,1}(74,:)'" : Constant  Value=[-0.290749364443431634885683934044209308922290802001953125;1.59300916003460368841615490964613854885101318359375;0.615546506145826288758371447329409420490264892578125;0.02933122821270021940431860230091842822730541229248046875;2.572654781445436356079881079494953155517578125;1.81191276559525515921222904580645263195037841796875]
      mask Display: e = 0.06;c1 = [120 150 230]/255;c2 = ([120 150 230]+0)/383;c3 = ([120 150 230]+128)/383;patch([0 1 1 0],[0 0 1 1],c1);patch([0 1 1 1-e 1-e 0+e],[0 0 1 1-e 0+e 0+e],c2);patch([0 0 1 1-e 0+e 0+e],[0 1 1 1-e 1-e 0+e],c3);plot([0 1 1 0 0],[0 0 1 1 0]);disp('Weights');
  "IW{1,1}(75,:)'" : Constant  Value=[-2.13164130554682795803955741575919091701507568359375;0.556137980375412066536000565974973142147064208984375;-0.401839179168786142515301662569981999695301055908203125;-2.434881976425903093996794268605299293994903564453125;-0.12120050356726909390747692896184162236750125885009765625;0.73568313356140013770101404588785953819751739501953125]
      mask Display: e = 0.06;c1 = [120 150 230]/255;c2 = ([120 150 230]+0)/383;c3 = ([120 150 230]+128)/383;patch([0 1 1 0],[0 0 1 1],c1);patch([0 1 1 1-e 1-e 0+e],[0 0 1 1-e 0+e 0+e],c2);patch([0 0 1 1-e 0+e 0+e],[0 1 1 1-e 1-e 0+e],c3);plot([0 1 1 0 0],[0 0 1 1 0]);disp('Weights');
  "IW{1,1}(76,:)'" : Constant  Value=[-0.408884077131765000245877672568894922733306884765625;-1.121860368170075172855604250798933207988739013671875;-2.4515265098438163704486214555799961090087890625;-1.9561983482951561530427397883613593876361846923828125;0.1562145061721324779124842052624444477260112762451171875;-0.440152998112042725953330091215320862829685211181640625]
      mask Display: e = 0.06;c1 = [120 150 230]/255;c2 = ([120 150 230]+0)/383;c3 = ([120 150 230]+128)/383;patch([0 1 1 0],[0 0 1 1],c1);patch([0 1 1 1-e 1-e 0+e],[0 0 1 1-e 0+e 0+e],c2);patch([0 0 1 1-e 0+e 0+e],[0 1 1 1-e 1-e 0+e],c3);plot([0 1 1 0 0],[0 0 1 1 0]);disp('Weights');
  "IW{1,1}(77,:)'" : Constant  Value=[1.084670287332844207384141554939560592174530029296875;-2.06651794370801411560023552738130092620849609375;0.052186812262794590733250288394629023969173431396484375;-2.28982400704278621361709156190045177936553955078125;0.88258835716460648512793341069482266902923583984375;0.70694745441204442926164119853638112545013427734375]
      mask Display: e = 0.06;c1 = [120 150 230]/255;c2 = ([120 150 230]+0)/383;c3 = ([120 150 230]+128)/383;patch([0 1 1 0],[0 0 1 1],c1);patch([0 1 1 1-e 1-e 0+e],[0 0 1 1-e 0+e 0+e],c2);patch([0 0 1 1-e 0+e 0+e],[0 1 1 1-e 1-e 0+e],c3);plot([0 1 1 0 0],[0 0 1 1 0]);disp('Weights');
  "IW{1,1}(78,:)'" : Constant  Value=[1.804994953768887189227143608150072395801544189453125;0.08994801983798261790781225499813444912433624267578125;-2.12539449453052942118347345967777073383331298828125;-0.6338316616559300786803987648454494774341583251953125;-1.780068761675720256931754192919470369815826416015625;-0.3277580908617461208365284619503654539585113525390625]
      mask Display: e = 0.06;c1 = [120 150 230]/255;c2 = ([120 150 230]+0)/383;c3 = ([120 150 230]+128)/383;patch([0 1 1 0],[0 0 1 1],c1);patch([0 1 1 1-e 1-e 0+e],[0 0 1 1-e 0+e 0+e],c2);patch([0 0 1 1-e 0+e 0+e],[0 1 1 1-e 1-e 0+e],c3);plot([0 1 1 0 0],[0 0 1 1 0]);disp('Weights');
  "IW{1,1}(79,:)'" : Constant  Value=[-1.1267126631536179548476184208993799984455108642578125;-1.0190704253438143123133841072558425366878509521484375;-2.098134347457654147461880711489357054233551025390625;-1.130599021510132029533224340411834418773651123046875;-1.7829530548665413203224261451396159827709197998046875;-0.9788798598040380216644962274585850536823272705078125]
      mask Display: e = 0.06;c1 = [120 150 230]/255;c2 = ([120 150 230]+0)/383;c3 = ([120 150 230]+128)/383;patch([0 1 1 0],[0 0 1 1],c1);patch([0 1 1 1-e 1-e 0+e],[0 0 1 1-e 0+e 0+e],c2);patch([0 0 1 1-e 0+e 0+e],[0 1 1 1-e 1-e 0+e],c3);plot([0 1 1 0 0],[0 0 1 1 0]);disp('Weights');
  "IW{1,1}(8,:)'" : Constant  Value=[2.047842020107324412236948774079792201519012451171875;0.81782902354840925074341839717817492783069610595703125;-1.9654187907182691930074724950827658176422119140625;1.386761746205301459866632285411469638347625732421875;0.81502596112361391789136177976615726947784423828125;0.4185743290592600640565024150419048964977264404296875]
      mask Display: e = 0.06;c1 = [120 150 230]/255;c2 = ([120 150 230]+0)/383;c3 = ([120 150 230]+128)/383;patch([0 1 1 0],[0 0 1 1],c1);patch([0 1 1 1-e 1-e 0+e],[0 0 1 1-e 0+e 0+e],c2);patch([0 0 1 1-e 0+e 0+e],[0 1 1 1-e 1-e 0+e],c3);plot([0 1 1 0 0],[0 0 1 1 0]);disp('Weights');
  "IW{1,1}(80,:)'" : Constant  Value=[1.84927754154137868880525275017134845256805419921875;1.2882506352737355115323225618340075016021728515625;0.459652445557766020645118487664149142801761627197265625;-2.225432815294698940533635322935879230499267578125;-0.2431761856359662410387301179071073420345783233642578125;1.1322634880665274348388038561097346246242523193359375]
      mask Display: e = 0.06;c1 = [120 150 230]/255;c2 = ([120 150 230]+0)/383;c3 = ([120 150 230]+128)/383;patch([0 1 1 0],[0 0 1 1],c1);patch([0 1 1 1-e 1-e 0+e],[0 0 1 1-e 0+e 0+e],c2);patch([0 0 1 1-e 0+e 0+e],[0 1 1 1-e 1-e 0+e],c3);plot([0 1 1 0 0],[0 0 1 1 0]);disp('Weights');
  "IW{1,1}(81,:)'" : Constant  Value=[0.940118003027538673421759085613302886486053466796875;-2.222274153229202742210190990590490400791168212890625;1.1360850907585733349236534195370040833950042724609375;0.830869144121889835474803476245142519474029541015625;-1.0187222195133986968329509181785397231578826904296875;1.688160716638612779405548280919902026653289794921875]
      mask Display: e = 0.06;c1 = [120 150 230]/255;c2 = ([120 150 230]+0)/383;c3 = ([120 150 230]+128)/383;patch([0 1 1 0],[0 0 1 1],c1);patch([0 1 1 1-e 1-e 0+e],[0 0 1 1-e 0+e 0+e],c2);patch([0 0 1 1-e 0+e 0+e],[0 1 1 1-e 1-e 0+e],c3);plot([0 1 1 0 0],[0 0 1 1 0]);disp('Weights');
  "IW{1,1}(82,:)'" : Constant  Value=[1.1000778035312190894501327420584857463836669921875;0.292219217619925031304006779464543797075748443603515625;-1.6885423669657930734189221766428090631961822509765625;0.045014949029452626383385194230868364684283733367919921875;2.178923106565709755244597545242868363857269287109375;1.7253800679542312668246495377388782799243927001953125]
      mask Display: e = 0.06;c1 = [120 150 230]/255;c2 = ([120 150 230]+0)/383;c3 = ([120 150 230]+128)/383;patch([0 1 1 0],[0 0 1 1],c1);patch([0 1 1 1-e 1-e 0+e],[0 0 1 1-e 0+e 0+e],c2);patch([0 0 1 1-e 0+e 0+e],[0 1 1 1-e 1-e 0+e],c3);plot([0 1 1 0 0],[0 0 1 1 0]);disp('Weights');
  "IW{1,1}(83,:)'" : Constant  Value=[-0.64475092099213882068653447277029044926166534423828125;1.0441888077512764265719624745543114840984344482421875;1.72784939706293361183497836464084684848785400390625;2.1708139626010183320659052697010338306427001953125;-0.0403454962398413774504746243110275827348232269287109375;-1.4658020428224742826017745755962096154689788818359375]
      mask Display: e = 0.06;c1 = [120 150 230]/255;c2 = ([120 150 230]+0)/383;c3 = ([120 150 230]+128)/383;patch([0 1 1 0],[0 0 1 1],c1);patch([0 1 1 1-e 1-e 0+e],[0 0 1 1-e 0+e 0+e],c2);patch([0 0 1 1-e 0+e 0+e],[0 1 1 1-e 1-e 0+e],c3);plot([0 1 1 0 0],[0 0 1 1 0]);disp('Weights');
  "IW{1,1}(84,:)'" : Constant  Value=[1.4736068582386234737668928573839366436004638671875;1.2678598679887767008978016747278161346912384033203125;-1.0857237326506765651146224627154879271984100341796875;-2.146310916240597332915740480530075728893280029296875;0.58511085625251679775971069830120541155338287353515625;1.3424384943949234649807067398796789348125457763671875]
      mask Display: e = 0.06;c1 = [120 150 230]/255;c2 = ([120 150 230]+0)/383;c3 = ([120 150 230]+128)/383;patch([0 1 1 0],[0 0 1 1],c1);patch([0 1 1 1-e 1-e 0+e],[0 0 1 1-e 0+e 0+e],c2);patch([0 0 1 1-e 0+e 0+e],[0 1 1 1-e 1-e 0+e],c3);plot([0 1 1 0 0],[0 0 1 1 0]);disp('Weights');
  "IW{1,1}(85,:)'" : Constant  Value=[0.79513414683936634030914092363673262298107147216796875;-0.404632680618792928139981768254074268043041229248046875;1.297506907812026266668681273586116731166839599609375;-1.3300413166329636549534143341588787734508514404296875;-2.618983860995188539533273797133006155490875244140625;-0.5825766626646231571839962271042168140411376953125]
      mask Display: e = 0.06;c1 = [120 150 230]/255;c2 = ([120 150 230]+0)/383;c3 = ([120 150 230]+128)/383;patch([0 1 1 0],[0 0 1 1],c1);patch([0 1 1 1-e 1-e 0+e],[0 0 1 1-e 0+e 0+e],c2);patch([0 0 1 1-e 0+e 0+e],[0 1 1 1-e 1-e 0+e],c3);plot([0 1 1 0 0],[0 0 1 1 0]);disp('Weights');
  "IW{1,1}(86,:)'" : Constant  Value=[1.8497809662423974064182630172581411898136138916015625;-1.411237747685833543442868176498450338840484619140625;-1.943130025718176501214884410728700459003448486328125;-0.47133932488242702429914743333938531577587127685546875;1.38063239002331616944729830720461905002593994140625;-0.427186677184749508118244420984410680830478668212890625]
      mask Display: e = 0.06;c1 = [120 150 230]/255;c2 = ([120 150 230]+0)/383;c3 = ([120 150 230]+128)/383;patch([0 1 1 0],[0 0 1 1],c1);patch([0 1 1 1-e 1-e 0+e],[0 0 1 1-e 0+e 0+e],c2);patch([0 0 1 1-e 0+e 0+e],[0 1 1 1-e 1-e 0+e],c3);plot([0 1 1 0 0],[0 0 1 1 0]);disp('Weights');
  "IW{1,1}(87,:)'" : Constant  Value=[-2.195997672633074326853375168866477906703948974609375;-1.6068203389931416946723174987710081040859222412109375;0.12033283680952326644142402756187948398292064666748046875;-0.9451813001175295436695478201727382838726043701171875;-1.3010850538627207750863590263179503381252288818359375;1.2421132031492516656356883686385117471218109130859375]
      mask Display: e = 0.06;c1 = [120 150 230]/255;c2 = ([120 150 230]+0)/383;c3 = ([120 150 230]+128)/383;patch([0 1 1 0],[0 0 1 1],c1);patch([0 1 1 1-e 1-e 0+e],[0 0 1 1-e 0+e 0+e],c2);patch([0 0 1 1-e 0+e 0+e],[0 1 1 1-e 1-e 0+e],c3);plot([0 1 1 0 0],[0 0 1 1 0]);disp('Weights');
  "IW{1,1}(88,:)'" : Constant  Value=[-2.066643656477146873129413506831042468547821044921875;-0.784350163250612464338473728275857865810394287109375;-1.2654354727956020898460565149434842169284820556640625;0.2656037982666143992815932506346143782138824462890625;0.82225514286400891439399174487334676086902618408203125;2.055601063679134643535917348344810307025909423828125]
      mask Display: e = 0.06;c1 = [120 150 230]/255;c2 = ([120 150 230]+0)/383;c3 = ([120 150 230]+128)/383;patch([0 1 1 0],[0 0 1 1],c1);patch([0 1 1 1-e 1-e 0+e],[0 0 1 1-e 0+e 0+e],c2);patch([0 0 1 1-e 0+e 0+e],[0 1 1 1-e 1-e 0+e],c3);plot([0 1 1 0 0],[0 0 1 1 0]);disp('Weights');
  "IW{1,1}(89,:)'" : Constant  Value=[-2.87418896478965280039119534194469451904296875;-0.7290390756987383813481073957518674433231353759765625;-0.05167809429476298566097369757699198089540004730224609375;-0.204148781204436746694597104578861035406589508056640625;0.9351748963589499030746310381800867617130279541015625;1.36082778833926010264576689223758876323699951171875]
      mask Display: e = 0.06;c1 = [120 150 230]/255;c2 = ([120 150 230]+0)/383;c3 = ([120 150 230]+128)/383;patch([0 1 1 0],[0 0 1 1],c1);patch([0 1 1 1-e 1-e 0+e],[0 0 1 1-e 0+e 0+e],c2);patch([0 0 1 1-e 0+e 0+e],[0 1 1 1-e 1-e 0+e],c3);plot([0 1 1 0 0],[0 0 1 1 0]);disp('Weights');
  "IW{1,1}(9,:)'" : Constant  Value=[2.365781451365563281541426476906053721904754638671875;0.6854304018517443086722096268204040825366973876953125;0.96575450517044625353690889824065379798412322998046875;-1.427341894630035579183413574355654418468475341796875;0.90116132952600447314495113459997810423374176025390625;-1.439882390403305567616598636959679424762725830078125]
      mask Display: e = 0.06;c1 = [120 150 230]/255;c2 = ([120 150 230]+0)/383;c3 = ([120 150 230]+128)/383;patch([0 1 1 0],[0 0 1 1],c1);patch([0 1 1 1-e 1-e 0+e],[0 0 1 1-e 0+e 0+e],c2);patch([0 0 1 1-e 0+e 0+e],[0 1 1 1-e 1-e 0+e],c3);plot([0 1 1 0 0],[0 0 1 1 0]);disp('Weights');
  "IW{1,1}(90,:)'" : Constant  Value=[2.399453192270857737611322590964846312999725341796875;-1.2959418716017629957804047080571763217449188232421875;-0.0253204205368434652478892843419089331291615962982177734375;1.983831899442054069737650934257544577121734619140625;0.40225511785114631546633745529106818139553070068359375;-0.128565659344537730479629544788622297346591949462890625]
      mask Display: e = 0.06;c1 = [120 150 230]/255;c2 = ([120 150 230]+0)/383;c3 = ([120 150 230]+128)/383;patch([0 1 1 0],[0 0 1 1],c1);patch([0 1 1 1-e 1-e 0+e],[0 0 1 1-e 0+e 0+e],c2);patch([0 0 1 1-e 0+e 0+e],[0 1 1 1-e 1-e 0+e],c3);plot([0 1 1 0 0],[0 0 1 1 0]);disp('Weights');
  "IW{1,1}(91,:)'" : Constant  Value=[-1.9016169028495628623431912274099886417388916015625;-1.354597547502867538327109286910854279994964599609375;0.09479424047339080061647109687328338623046875;1.0643705725916225990346219987259246408939361572265625;1.2204046864633044666703654002049006521701812744140625;1.8083591840516370918834354597493074834346771240234375]
      mask Display: e = 0.06;c1 = [120 150 230]/255;c2 = ([120 150 230]+0)/383;c3 = ([120 150 230]+128)/383;patch([0 1 1 0],[0 0 1 1],c1);patch([0 1 1 1-e 1-e 0+e],[0 0 1 1-e 0+e 0+e],c2);patch([0 0 1 1-e 0+e 0+e],[0 1 1 1-e 1-e 0+e],c3);plot([0 1 1 0 0],[0 0 1 1 0]);disp('Weights');
  "IW{1,1}(92,:)'" : Constant  Value=[-0.87893811393256127129092192262760363519191741943359375;0.364530303677403300088855075955507345497608184814453125;1.511590208708633920053898691548965871334075927734375;0.83839521783053327919077446495066396892070770263671875;2.304796035048912283826894054072909057140350341796875;-1.6278788153528740423325871233828365802764892578125]
      mask Display: e = 0.06;c1 = [120 150 230]/255;c2 = ([120 150 230]+0)/383;c3 = ([120 150 230]+128)/383;patch([0 1 1 0],[0 0 1 1],c1);patch([0 1 1 1-e 1-e 0+e],[0 0 1 1-e 0+e 0+e],c2);patch([0 0 1 1-e 0+e 0+e],[0 1 1 1-e 1-e 0+e],c3);plot([0 1 1 0 0],[0 0 1 1 0]);disp('Weights');
  "IW{1,1}(93,:)'" : Constant  Value=[-0.48553762366738684175260232223081402480602264404296875;0.87980812442820843788382489947252906858921051025390625;1.5814295662891233451574635182623751461505889892578125;-0.10003432900378328440638142637908458709716796875;2.503689178757091848837035286123864352703094482421875;1.4182497406725691480033901825663633644580841064453125]
      mask Display: e = 0.06;c1 = [120 150 230]/255;c2 = ([120 150 230]+0)/383;c3 = ([120 150 230]+128)/383;patch([0 1 1 0],[0 0 1 1],c1);patch([0 1 1 1-e 1-e 0+e],[0 0 1 1-e 0+e 0+e],c2);patch([0 0 1 1-e 0+e 0+e],[0 1 1 1-e 1-e 0+e],c3);plot([0 1 1 0 0],[0 0 1 1 0]);disp('Weights');
  "IW{1,1}(94,:)'" : Constant  Value=[2.803508575759152687822961524943821132183074951171875;-0.0212162892076034094446246314191739656962454319000244140625;0.7204785757559903913715970702469348907470703125;-0.2142528507395309034233576994665781967341899871826171875;1.357673981613794378375814630999229848384857177734375;-1.1174916158345749028768523203325457870960235595703125]
      mask Display: e = 0.06;c1 = [120 150 230]/255;c2 = ([120 150 230]+0)/383;c3 = ([120 150 230]+128)/383;patch([0 1 1 0],[0 0 1 1],c1);patch([0 1 1 1-e 1-e 0+e],[0 0 1 1-e 0+e 0+e],c2);patch([0 0 1 1-e 0+e 0+e],[0 1 1 1-e 1-e 0+e],c3);plot([0 1 1 0 0],[0 0 1 1 0]);disp('Weights');
  "IW{1,1}(95,:)'" : Constant  Value=[2.167879180123545523883876740001142024993896484375;-0.853157853774927144030471026781015098094940185546875;1.7469402706615593245942363864742219448089599609375;0.026219799132155309495662010021987953223288059234619140625;1.1264612512380380859866590981255285441875457763671875;-1.4063449819091446979513193582533858716487884521484375]
      mask Display: e = 0.06;c1 = [120 150 230]/255;c2 = ([120 150 230]+0)/383;c3 = ([120 150 230]+128)/383;patch([0 1 1 0],[0 0 1 1],c1);patch([0 1 1 1-e 1-e 0+e],[0 0 1 1-e 0+e 0+e],c2);patch([0 0 1 1-e 0+e 0+e],[0 1 1 1-e 1-e 0+e],c3);plot([0 1 1 0 0],[0 0 1 1 0]);disp('Weights');
  "IW{1,1}(96,:)'" : Constant  Value=[-1.90426963744236044107083216658793389797210693359375;0.86127963943865648577258298246306367218494415283203125;1.1635172068365686737223541058483533561229705810546875;-0.87935694329516655987077911049709655344486236572265625;1.6856508765391506887709738293779082596302032470703125;1.4663138990901256608623270949465222656726837158203125]
      mask Display: e = 0.06;c1 = [120 150 230]/255;c2 = ([120 150 230]+0)/383;c3 = ([120 150 230]+128)/383;patch([0 1 1 0],[0 0 1 1],c1);patch([0 1 1 1-e 1-e 0+e],[0 0 1 1-e 0+e 0+e],c2);patch([0 0 1 1-e 0+e 0+e],[0 1 1 1-e 1-e 0+e],c3);plot([0 1 1 0 0],[0 0 1 1 0]);disp('Weights');
  "IW{1,1}(97,:)'" : Constant  Value=[-0.386563792318184329399599619137006811797618865966796875;1.5146650280141733535543835387215949594974517822265625;-1.678492864441452514512320703943260014057159423828125;1.6768959077438221338951507277670316398143768310546875;0.8136987648699680608643802770529873669147491455078125;1.7032649272001361140382869052700698375701904296875]
      mask Display: e = 0.06;c1 = [120 150 230]/255;c2 = ([120 150 230]+0)/383;c3 = ([120 150 230]+128)/383;patch([0 1 1 0],[0 0 1 1],c1);patch([0 1 1 1-e 1-e 0+e],[0 0 1 1-e 0+e 0+e],c2);patch([0 0 1 1-e 0+e 0+e],[0 1 1 1-e 1-e 0+e],c3);plot([0 1 1 0 0],[0 0 1 1 0]);disp('Weights');
  "IW{1,1}(98,:)'" : Constant  Value=[-1.2409933121580898340852172623272053897380828857421875;1.587808809971514190095831509097479283809661865234375;-2.072404457400150334933641715906560420989990234375;0.86681046818774376561123062856495380401611328125;-0.7999511695856560411499458496109582483768463134765625;1.247706313942196221233871256117708981037139892578125]
      mask Display: e = 0.06;c1 = [120 150 230]/255;c2 = ([120 150 230]+0)/383;c3 = ([120 150 230]+128)/383;patch([0 1 1 0],[0 0 1 1],c1);patch([0 1 1 1-e 1-e 0+e],[0 0 1 1-e 0+e 0+e],c2);patch([0 0 1 1-e 0+e 0+e],[0 1 1 1-e 1-e 0+e],c3);plot([0 1 1 0 0],[0 0 1 1 0]);disp('Weights');
  "IW{1,1}(99,:)'" : Constant  Value=[-1.4073673028966176001830490349675528705120086669921875;1.4956345625709719371343453531153500080108642578125;1.295359737224632823426873073913156986236572265625;1.540897519490569411715341630042530596256256103515625;0.1579760996919972459995307190183666534721851348876953125;1.7818237993087657766722031738026998937129974365234375]
      mask Display: e = 0.06;c1 = [120 150 230]/255;c2 = ([120 150 230]+0)/383;c3 = ([120 150 230]+128)/383;patch([0 1 1 0],[0 0 1 1],c1);patch([0 1 1 1-e 1-e 0+e],[0 0 1 1-e 0+e 0+e],c2);patch([0 0 1 1-e 0+e 0+e],[0 1 1 1-e 1-e 0+e],c3);plot([0 1 1 0 0],[0 0 1 1 0]);disp('Weights');
  Mux : Mux  Inputs=200
      mask Display: e = 0.06;c1 = [120 150 230]/255;c2 = ([120 150 230]+0)/383;c3 = ([120 150 230]+128)/383;patch([0 1 1 0],[0 0 1 1],c1);patch([0 1 1 1-e 1-e 0+e],[0 0 1 1-e 0+e 0+e],c2);patch([0 0 1 1-e 0+e 0+e],[0 1 1 1-e 1-e 0+e],c3);plot([0 1 1 0 0],[0 0 1 1 0]);disp('Mux');
  dotprod{1..200} (200 alike) : neural/Weight Functions/dotprod
  "iz{1,1}" : Outport
      mask Display: e = 0.06;c1 = [120 230 180]/255;c2 = ([120 230 180]+0)/(256+128);c3 = ([120 230 180]+128)/(256+128);patch([0 1 1 0],[0 0 1 1],c1);patch([0 1 1 1-e 1-e 0+e],[0 0 1 1-e 0+e 0+e],c2);patch([0 0 1 1-e 0+e 0+e],[0 1 1 1-e 1-e 0+e],c3);plot([0 1 1 0 0],[0 0 1 1 0]);
  wires:
  "IW{1,1}(1,:)'"/1 -> dotprod1/1
  "pd{1,1}"/1 -> dotprod1/2, dotprod2/2, dotprod3/2, dotprod4/2, dotprod5/2, dotprod6/2, dotprod7/2, dotprod8/2, dotprod9/2, dotprod10/2, dotprod11/2, dotprod12/2, dotprod13/2, dotprod14/2, dotprod15/2, dotprod16/2, dotprod17/2, dotprod18/2, dotprod19/2, dotprod20/2, dotprod21/2, dotprod22/2, dotprod23/2, dotprod24/2, dotprod25/2, dotprod26/2, dotprod27/2, dotprod28/2, dotprod29/2, dotprod30/2, dotprod31/2, dotprod32/2, dotprod33/2, dotprod34/2, dotprod35/2, dotprod36/2, dotprod37/2, dotprod38/2, dotprod39/2, dotprod40/2, dotprod41/2, dotprod42/2, dotprod43/2, dotprod44/2, dotprod45/2, dotprod46/2, dotprod47/2, dotprod48/2, dotprod49/2, dotprod50/2, dotprod51/2, dotprod52/2, dotprod53/2, dotprod54/2, dotprod55/2, dotprod56/2, dotprod57/2, dotprod58/2, dotprod59/2, dotprod60/2, dotprod61/2, dotprod62/2, dotprod63/2, dotprod64/2, dotprod65/2, dotprod66/2, dotprod67/2, dotprod68/2, dotprod69/2, dotprod70/2, dotprod71/2, dotprod72/2, dotprod73/2, dotprod74/2, dotprod75/2, dotprod76/2, dotprod77/2, dotprod78/2, dotprod79/2, dotprod80/2, dotprod81/2, dotprod82/2, dotprod83/2, dotprod84/2, dotprod85/2, dotprod86/2, dotprod87/2, dotprod88/2, dotprod89/2, dotprod90/2, dotprod91/2, dotprod92/2, dotprod93/2, dotprod94/2, dotprod95/2, dotprod96/2, dotprod97/2, dotprod98/2, dotprod99/2, dotprod100/2, dotprod101/2, dotprod102/2, dotprod103/2, dotprod104/2, dotprod105/2, dotprod106/2, dotprod107/2, dotprod108/2, dotprod109/2, dotprod110/2, dotprod111/2, dotprod112/2, dotprod113/2, dotprod114/2, dotprod115/2, dotprod116/2, dotprod117/2, dotprod118/2, dotprod119/2, dotprod120/2, dotprod121/2, dotprod122/2, dotprod123/2, dotprod124/2, dotprod125/2, dotprod126/2, dotprod127/2, dotprod128/2, dotprod129/2, dotprod130/2, dotprod131/2, dotprod132/2, dotprod133/2, dotprod134/2, dotprod135/2, dotprod136/2, dotprod137/2, dotprod138/2, dotprod139/2, dotprod140/2, dotprod141/2, dotprod142/2, dotprod143/2, dotprod144/2, dotprod145/2, dotprod146/2, dotprod147/2, dotprod148/2, dotprod149/2, dotprod150/2, dotprod151/2, dotprod152/2, dotprod153/2, dotprod154/2, dotprod155/2, dotprod156/2, dotprod157/2, dotprod158/2, dotprod159/2, dotprod160/2, dotprod161/2, dotprod162/2, dotprod163/2, dotprod164/2, dotprod165/2, dotprod166/2, dotprod167/2, dotprod168/2, dotprod169/2, dotprod170/2, dotprod171/2, dotprod172/2, dotprod173/2, dotprod174/2, dotprod175/2, dotprod176/2, dotprod177/2, dotprod178/2, dotprod179/2, dotprod180/2, dotprod181/2, dotprod182/2, dotprod183/2, dotprod184/2, dotprod185/2, dotprod186/2, dotprod187/2, dotprod188/2, dotprod189/2, dotprod190/2, dotprod191/2, dotprod192/2, dotprod193/2, dotprod194/2, dotprod195/2, dotprod196/2, dotprod197/2, dotprod198/2, dotprod199/2, dotprod200/2
  dotprod1/1 -> Mux/1
  "IW{1,1}(2,:)'"/1 -> dotprod2/1
  dotprod2/1 -> Mux/2
  "IW{1,1}(3,:)'"/1 -> dotprod3/1
  dotprod3/1 -> Mux/3
  "IW{1,1}(4,:)'"/1 -> dotprod4/1
  dotprod4/1 -> Mux/4
  "IW{1,1}(5,:)'"/1 -> dotprod5/1
  dotprod5/1 -> Mux/5
  "IW{1,1}(6,:)'"/1 -> dotprod6/1
  dotprod6/1 -> Mux/6
  "IW{1,1}(7,:)'"/1 -> dotprod7/1
  dotprod7/1 -> Mux/7
  "IW{1,1}(8,:)'"/1 -> dotprod8/1
  dotprod8/1 -> Mux/8
  "IW{1,1}(9,:)'"/1 -> dotprod9/1
  dotprod9/1 -> Mux/9
  "IW{1,1}(10,:)'"/1 -> dotprod10/1
  dotprod10/1 -> Mux/10
  "IW{1,1}(11,:)'"/1 -> dotprod11/1
  dotprod11/1 -> Mux/11
  "IW{1,1}(12,:)'"/1 -> dotprod12/1
  dotprod12/1 -> Mux/12
  "IW{1,1}(13,:)'"/1 -> dotprod13/1
  dotprod13/1 -> Mux/13
  "IW{1,1}(14,:)'"/1 -> dotprod14/1
  dotprod14/1 -> Mux/14
  "IW{1,1}(15,:)'"/1 -> dotprod15/1
  dotprod15/1 -> Mux/15
  "IW{1,1}(16,:)'"/1 -> dotprod16/1
  dotprod16/1 -> Mux/16
  "IW{1,1}(17,:)'"/1 -> dotprod17/1
  dotprod17/1 -> Mux/17
  "IW{1,1}(18,:)'"/1 -> dotprod18/1
  dotprod18/1 -> Mux/18
  "IW{1,1}(19,:)'"/1 -> dotprod19/1
  dotprod19/1 -> Mux/19
  "IW{1,1}(20,:)'"/1 -> dotprod20/1
  dotprod20/1 -> Mux/20
  "IW{1,1}(21,:)'"/1 -> dotprod21/1
  dotprod21/1 -> Mux/21
  "IW{1,1}(22,:)'"/1 -> dotprod22/1
  dotprod22/1 -> Mux/22
  "IW{1,1}(23,:)'"/1 -> dotprod23/1
  dotprod23/1 -> Mux/23
  "IW{1,1}(24,:)'"/1 -> dotprod24/1
  dotprod24/1 -> Mux/24
  "IW{1,1}(25,:)'"/1 -> dotprod25/1
  dotprod25/1 -> Mux/25
  "IW{1,1}(26,:)'"/1 -> dotprod26/1
  dotprod26/1 -> Mux/26
  "IW{1,1}(27,:)'"/1 -> dotprod27/1
  dotprod27/1 -> Mux/27
  "IW{1,1}(28,:)'"/1 -> dotprod28/1
  dotprod28/1 -> Mux/28
  "IW{1,1}(29,:)'"/1 -> dotprod29/1
  dotprod29/1 -> Mux/29
  "IW{1,1}(30,:)'"/1 -> dotprod30/1
  dotprod30/1 -> Mux/30
  "IW{1,1}(31,:)'"/1 -> dotprod31/1
  dotprod31/1 -> Mux/31
  "IW{1,1}(32,:)'"/1 -> dotprod32/1
  dotprod32/1 -> Mux/32
  "IW{1,1}(33,:)'"/1 -> dotprod33/1
  dotprod33/1 -> Mux/33
  "IW{1,1}(34,:)'"/1 -> dotprod34/1
  dotprod34/1 -> Mux/34
  "IW{1,1}(35,:)'"/1 -> dotprod35/1
  dotprod35/1 -> Mux/35
  "IW{1,1}(36,:)'"/1 -> dotprod36/1
  dotprod36/1 -> Mux/36
  "IW{1,1}(37,:)'"/1 -> dotprod37/1
  dotprod37/1 -> Mux/37
  "IW{1,1}(38,:)'"/1 -> dotprod38/1
  dotprod38/1 -> Mux/38
  "IW{1,1}(39,:)'"/1 -> dotprod39/1
  dotprod39/1 -> Mux/39
  "IW{1,1}(40,:)'"/1 -> dotprod40/1
  dotprod40/1 -> Mux/40
  "IW{1,1}(41,:)'"/1 -> dotprod41/1
  dotprod41/1 -> Mux/41
  "IW{1,1}(42,:)'"/1 -> dotprod42/1
  dotprod42/1 -> Mux/42
  "IW{1,1}(43,:)'"/1 -> dotprod43/1
  dotprod43/1 -> Mux/43
  "IW{1,1}(44,:)'"/1 -> dotprod44/1
  dotprod44/1 -> Mux/44
  "IW{1,1}(45,:)'"/1 -> dotprod45/1
  dotprod45/1 -> Mux/45
  "IW{1,1}(46,:)'"/1 -> dotprod46/1
  dotprod46/1 -> Mux/46
  "IW{1,1}(47,:)'"/1 -> dotprod47/1
  dotprod47/1 -> Mux/47
  "IW{1,1}(48,:)'"/1 -> dotprod48/1
  dotprod48/1 -> Mux/48
  "IW{1,1}(49,:)'"/1 -> dotprod49/1
  dotprod49/1 -> Mux/49
  "IW{1,1}(50,:)'"/1 -> dotprod50/1
  dotprod50/1 -> Mux/50
  "IW{1,1}(51,:)'"/1 -> dotprod51/1
  dotprod51/1 -> Mux/51
  "IW{1,1}(52,:)'"/1 -> dotprod52/1
  dotprod52/1 -> Mux/52
  "IW{1,1}(53,:)'"/1 -> dotprod53/1
  dotprod53/1 -> Mux/53
  "IW{1,1}(54,:)'"/1 -> dotprod54/1
  dotprod54/1 -> Mux/54
  "IW{1,1}(55,:)'"/1 -> dotprod55/1
  dotprod55/1 -> Mux/55
  "IW{1,1}(56,:)'"/1 -> dotprod56/1
  dotprod56/1 -> Mux/56
  "IW{1,1}(57,:)'"/1 -> dotprod57/1
  dotprod57/1 -> Mux/57
  "IW{1,1}(58,:)'"/1 -> dotprod58/1
  dotprod58/1 -> Mux/58
  "IW{1,1}(59,:)'"/1 -> dotprod59/1
  dotprod59/1 -> Mux/59
  "IW{1,1}(60,:)'"/1 -> dotprod60/1
  dotprod60/1 -> Mux/60
  "IW{1,1}(61,:)'"/1 -> dotprod61/1
  dotprod61/1 -> Mux/61
  "IW{1,1}(62,:)'"/1 -> dotprod62/1
  dotprod62/1 -> Mux/62
  "IW{1,1}(63,:)'"/1 -> dotprod63/1
  dotprod63/1 -> Mux/63
  "IW{1,1}(64,:)'"/1 -> dotprod64/1
  dotprod64/1 -> Mux/64
  "IW{1,1}(65,:)'"/1 -> dotprod65/1
  dotprod65/1 -> Mux/65
  "IW{1,1}(66,:)'"/1 -> dotprod66/1
  dotprod66/1 -> Mux/66
  "IW{1,1}(67,:)'"/1 -> dotprod67/1
  dotprod67/1 -> Mux/67
  "IW{1,1}(68,:)'"/1 -> dotprod68/1
  dotprod68/1 -> Mux/68
  "IW{1,1}(69,:)'"/1 -> dotprod69/1
  dotprod69/1 -> Mux/69
  "IW{1,1}(70,:)'"/1 -> dotprod70/1
  dotprod70/1 -> Mux/70
  "IW{1,1}(71,:)'"/1 -> dotprod71/1
  dotprod71/1 -> Mux/71
  "IW{1,1}(72,:)'"/1 -> dotprod72/1
  dotprod72/1 -> Mux/72
  "IW{1,1}(73,:)'"/1 -> dotprod73/1
  dotprod73/1 -> Mux/73
  "IW{1,1}(74,:)'"/1 -> dotprod74/1
  dotprod74/1 -> Mux/74
  "IW{1,1}(75,:)'"/1 -> dotprod75/1
  dotprod75/1 -> Mux/75
  "IW{1,1}(76,:)'"/1 -> dotprod76/1
  dotprod76/1 -> Mux/76
  "IW{1,1}(77,:)'"/1 -> dotprod77/1
  dotprod77/1 -> Mux/77
  "IW{1,1}(78,:)'"/1 -> dotprod78/1
  dotprod78/1 -> Mux/78
  "IW{1,1}(79,:)'"/1 -> dotprod79/1
  dotprod79/1 -> Mux/79
  "IW{1,1}(80,:)'"/1 -> dotprod80/1
  dotprod80/1 -> Mux/80
